simulink model "35 Bus Network Electricity Transmission Model"  (R2023b)
settings: Solver=VariableStepAuto  StartTime=0.0  StopTime=1  RelTol=1e-3
model workspace (MAT data in the model file):
  T_set = 0.0001
  Tp = 5e-05
undefined symbols (not defined in the file): D1, D11, Delta, DiscIntNeverNeededParam
libraries: spsSeriesRLCBranchLib x57, spsLoadFlowBusLib x35, spsThreePhaseSeriesRLCLoadLib x28, spsThreePhaseTransformerTwoWindingsLib x22, spsDistributedParametersLineLib x22, spsGenericPowerSystemStabilizerLib x20, spsThreePhaseVIMeasurementLib x14, spsSynchronousMachinepuStandardLib x10, spsExcitationSystemLib x10, spsHydraulicTurbineandGovernorLib x10, spsFourierLib x8, spsMeanLib x8
(part 5 of 8)

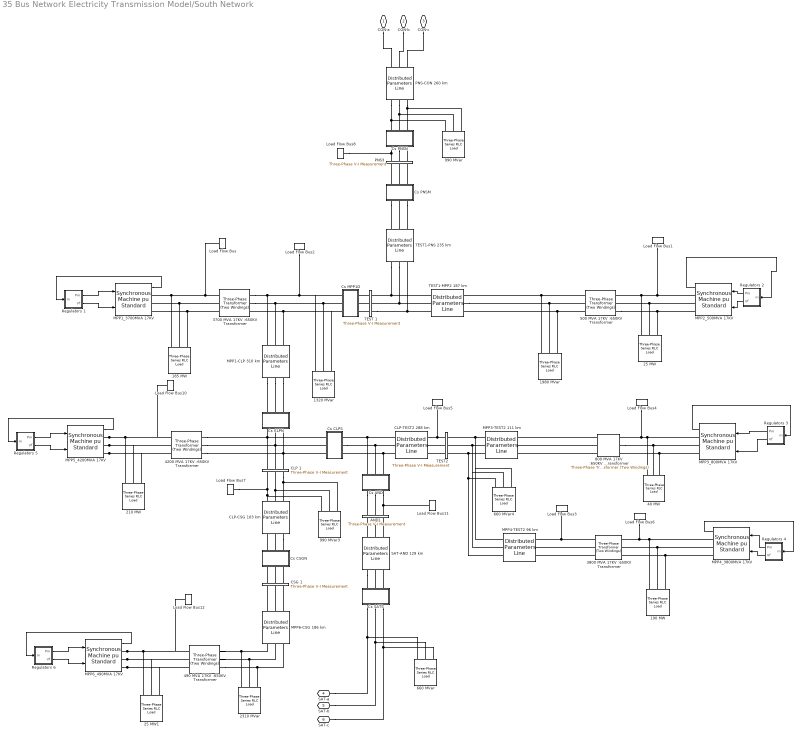
== system 35 Bus Network Electricity Transmission Model/South Network ==
  " SAT-AND 129 km" : spsDistributedParametersLineLib/Distributed Parameters Line  Phases=3  Length=129  Frequency=60  Resistance=[0.01273 0.3864]/6  Inductance="[0.9337e-3  4.1264e-3]/6"  Capacitance=[12.74e-9 7.751e-9]*6  x1=[-0.00078 2.90768445580107e-08 -136458.201500548 -192658.826474025;-0.00072 2.99535903710452e-08 -132065.820469422 -195695.922168478;-0.00066 3.08150113737671e-08 -127605.872124249 -198632.896213104;-0.0006 3.16606668472743e-08 -123080.638257011 -201468.245997714;-0.00054 3.24901241386005e-08 -118492.434060973 -204200.520904966;-0.00048 3.3302958882069e-08 -113843.60694618 -206828.323052531;-0.00042 3.40987552164055e-08 -109136.535338486 -209350.308008275;-0.00036 3.48771059975007e-08 -104373.627462701 -211765.185478092;-0.0003 3.56376130067127e-08 -99557.3201105034 -214071.719966049;-0.00024 3.63798871546032e-08 -94690.0773937295 -216268.73140648;-0.00018 3.71035486800023e-08 -89774.3894836895 -218355.095767737;-0.00012 3.7808227344302e-08 -84812.7713371497 -220329.745627261;-6e-05 3.84935626208767e-08 -79807.761409634 -222191.670717696]  x2=[-0.00078 6.20574629908019e-08 -60655.3196005387 -176454.698626756;-0.00072 6.44563826133641e-08 -56648.8312166304 -177781.461927132;-0.00066 6.68223251595644e-08 -52613.3602439216 -179017.268946562;-0.0006 6.91540801694784e-08 -48550.9713039289 -180161.487423341;-0.00054 7.14504546741573e-08 -44463.7427898983 -181213.531954152;-0.00048 7.37102738059722e-08 -40353.7658034608 -182172.864293574;-0.00042 7.59323813996988e-08 -36223.1430847865 -183038.993629456;-0.00036 7.81156405840321e-08 -32073.9879367833 -183811.476834026;-0.0003 8.02589343632316e-08 -27908.4231438924 -184489.918690602;-0.00024 8.23611661885963e-08 -23728.5798860328 -185073.972095794;-0.00018 8.44212605194795e-08 -19536.5966482498 -185563.338237088;-0.00012 8.64381633735555e-08 -15334.6181266266 -185957.766745723;-6e-05 8.84108428660558e-08 -11124.7941310188 -186257.055824787]  x3=[-0.00078 -1.45980787087981e-09 -866.244947874634 -13940.0125713573;-0.00072 -1.42091668020749e-09 -550.734822343354 -13956.0401157641;-0.00066 -1.38129852230606e-09 -234.942930700552 -13964.9274921696;-0.0006 -1.34097366655716e-09 80.9691620868421 -13966.670153628;-0.00054 -1.2999627439021e-09 396.839829554774 -13961.2672085614;-0.00048 -1.25828673628672e-09 712.50746643315 -13948.7214212164;-0.00042 -1.21596696592658e-09 1027.81057132607 -13929.0392102495;-0.00036 -1.17302508439819e-09 1342.58782933895 -13902.2306454436;-0.0003 -1.1294830615616e-09 1656.67819461017 -13868.3094425558;-0.00024 -1.08536317432028e-09 1969.92097270513 -13827.2929563003;-0.00018 -1.04068799522377e-09 2282.1559028305 -13779.2021714693;-0.00012 -9.95480380919198e-10 2593.22323982659 -13724.0616921971;-6e-05 -9.49763460457386e-10 2902.96383589593 -13661.8997293716]  x4=[-0.00078 2.00884929255157e-09 -4168.15373979615 6162.62143218946;-0.00072 1.99781306681485e-09 -4306.47032100265 6066.77150994181;-0.00066 1.9857547229978e-09 -4442.5836324185 5967.81771528863;-0.0006 1.97268043037194e-09 -4576.42403595849 5865.81067481971;-0.00054 1.95859687798696e-09 -4707.9230563991 5760.80257722184;-0.00048 1.94351127124849e-09 -4837.01341641164 5652.84714657807;-0.00042 1.92743132823169e-09 -4963.62907098261 5541.9996148815;-0.00036 1.91036527573254e-09 -5087.70524120354 5428.31669377758;-0.0003 1.89232184505882e-09 -5209.17844741309 5311.85654554936;-0.00024 1.87331026756309e-09 -5327.9865416744 5192.67875336062;-0.00018 1.85334026991968e-09 -5444.06873957111 5070.84429077198;-0.00012 1.83242206914838e-09 -5557.36565130583 4946.41549054576;-6e-05 1.81056636738724e-09 -5667.81931208504 4819.45601275533]  x5=0.000729548621424508  V1=[2.188e-18 3.182e-07 3.182e-07;377 377 377;0.6306 1.295 -0.2758]  V2=[1.209e-19 1.011e-07 1.011e-07;377 377 377;-2.255 -1.798 2.915]  I1=[1.016e-20 9.164e-09 9.164e-09;377 377 377;2.19 2.786 1.215]  I2=[1.089e-20 9.22e-09 9.22e-09;377 377 377;-0.7019 -0.2685 -1.839]  nHarmo=1  Measurements=None  Decoupling=off  VsMag0=0  VrMag0=0  VsAngle0=0  VrAngle0=0  IsMag0=0  IrMag0=0  IsAngle0=0  IrAngle0=0
      settings: LibrarySourceBlock=sps_lib/Power Grid Elements/Distributed Parameters Line
  1320 MVar : spsThreePhaseSeriesRLCLoadLib/Three-Phase Series RLC Load  LConnTagsString=A|B|C  Configuration=Y (grounded)  NominalVoltage=650e3  Vabc=[1e3 1e3 1e3]  Vabcp=[1e3 1e3 1e3]  NominalFrequency=60  UnbalancedPower=off  ActivePower=4400e3  InductivePower=1320e6  CapacitivePower=0  Pabc=[10e3 9e3 11e3]  QLabc=[100 90 110]  QCabc=[100 90 110]  Pabcp=[10e3 9e3 11e3]  QLabcp=[100 90 110]  QCabcp=[100 90 110]  Measurements=None  LoadType=constant Z
  185 MW : spsThreePhaseSeriesRLCLoadLib/Three-Phase Series RLC Load  LConnTagsString=A|B|C  Configuration=Y (grounded)  NominalVoltage=17e3  Vabc=[1e3 1e3 1e3]  Vabcp=[1e3 1e3 1e3]  NominalFrequency=60  UnbalancedPower=off  ActivePower=185e6  InductivePower=0  CapacitivePower=0  Pabc=[10e3 9e3 11e3]  QLabc=[100 90 110]  QCabc=[100 90 110]  Pabcp=[10e3 9e3 11e3]  QLabcp=[100 90 110]  QCabcp=[100 90 110]  Measurements=None  LoadType=constant Z
  190 MW : spsThreePhaseSeriesRLCLoadLib/Three-Phase Series RLC Load  LConnTagsString=A|B|C  Configuration=Y (grounded)  NominalVoltage=17e3  Vabc=[1e3 1e3 1e3]  Vabcp=[1e3 1e3 1e3]  NominalFrequency=60  UnbalancedPower=off  ActivePower=190e6  InductivePower=0  CapacitivePower=0  Pabc=[10e3 9e3 11e3]  QLabc=[100 90 110]  QCabc=[100 90 110]  Pabcp=[10e3 9e3 11e3]  QLabcp=[100 90 110]  QCabcp=[100 90 110]  Measurements=None  LoadType=constant Z
  1980 MVar : spsThreePhaseSeriesRLCLoadLib/Three-Phase Series RLC Load  LConnTagsString=A|B|C  Configuration=Y (grounded)  NominalVoltage=650e3  Vabc=[1e3 1e3 1e3]  Vabcp=[1e3 1e3 1e3]  NominalFrequency=60  UnbalancedPower=off  ActivePower=4400e3  InductivePower=1320e6  CapacitivePower=0  Pabc=[10e3 9e3 11e3]  QLabc=[100 90 110]  QCabc=[100 90 110]  Pabcp=[10e3 9e3 11e3]  QLabcp=[100 90 110]  QCabcp=[100 90 110]  Measurements=None  LoadType=constant Z
  210 MW : spsThreePhaseSeriesRLCLoadLib/Three-Phase Series RLC Load  LConnTagsString=A|B|C  Configuration=Y (grounded)  NominalVoltage=17e3  Vabc=[1e3 1e3 1e3]  Vabcp=[1e3 1e3 1e3]  NominalFrequency=60  UnbalancedPower=off  ActivePower=210e6  InductivePower=0  CapacitivePower=0  Pabc=[10e3 9e3 11e3]  QLabc=[100 90 110]  QCabc=[100 90 110]  Pabcp=[10e3 9e3 11e3]  QLabcp=[100 90 110]  QCabcp=[100 90 110]  Measurements=None  LoadType=constant Z
  2310 MVar : spsThreePhaseSeriesRLCLoadLib/Three-Phase Series RLC Load  LConnTagsString=A|B|C  Configuration=Y (grounded)  NominalVoltage=650e3  Vabc=[1e3 1e3 1e3]  Vabcp=[1e3 1e3 1e3]  NominalFrequency=60  UnbalancedPower=off  ActivePower=7700e3  InductivePower=2310e6  CapacitivePower=0  Pabc=[10e3 9e3 11e3]  QLabc=[100 90 110]  QCabc=[100 90 110]  Pabcp=[10e3 9e3 11e3]  QLabcp=[100 90 110]  QCabcp=[100 90 110]  Measurements=None  LoadType=constant Z
  25 MW : spsThreePhaseSeriesRLCLoadLib/Three-Phase Series RLC Load  LConnTagsString=A|B|C  Configuration=Y (grounded)  NominalVoltage=17e3  Vabc=[1e3 1e3 1e3]  Vabcp=[1e3 1e3 1e3]  NominalFrequency=60  UnbalancedPower=off  ActivePower=25e6  InductivePower=0  CapacitivePower=0  Pabc=[10e3 9e3 11e3]  QLabc=[100 90 110]  QCabc=[100 90 110]  Pabcp=[10e3 9e3 11e3]  QLabcp=[100 90 110]  QCabcp=[100 90 110]  Measurements=None  LoadType=constant Z
  25 MW1 : spsThreePhaseSeriesRLCLoadLib/Three-Phase Series RLC Load  LConnTagsString=A|B|C  Configuration=Y (grounded)  NominalVoltage=17e3  Vabc=[1e3 1e3 1e3]  Vabcp=[1e3 1e3 1e3]  NominalFrequency=60  UnbalancedPower=off  ActivePower=25e6  InductivePower=0  CapacitivePower=0  Pabc=[10e3 9e3 11e3]  QLabc=[100 90 110]  QCabc=[100 90 110]  Pabcp=[10e3 9e3 11e3]  QLabcp=[100 90 110]  QCabcp=[100 90 110]  Measurements=None  LoadType=constant Z
  "3700 MVA 17KV :650KV Transformer " : spsThreePhaseTransformerTwoWindingsLib/Three-Phase Transformer (Two Windings)  Winding1Connection=Delta (D1)  Winding2Connection=Yg  CoreType=Three single-phase transformers  SetSaturation=off  Hysteresis=off  DataFile='hysteresis'  SetInitialFlux=off  Measurements=None  UNITS=pu  NominalPower=[ 3700e6 , 60 ]  Winding1=[ 17e3 , 0.002 , 0.08 ]  Winding2=[ 650e3 , 0.002 , 0.08 ]  Rm=500  Lm=500  L0=0.5  Saturation=[ 0,0 ; 0.0024,1.2 ; 1.0,1.52 ]  InitialFluxes=[ 0.8 , -0.8 , 0.7 ]  BreakLoop=off  DiscreteSolver=Trapezoidal iterative  DataType=off  TransfoNumber=1
  3800 MVA 17KV :650KV Transformer : spsThreePhaseTransformerTwoWindingsLib/Three-Phase Transformer (Two Windings)  Winding1Connection=Yg  Winding2Connection=Delta (D1)  CoreType=Three single-phase transformers  SetSaturation=off  Hysteresis=off  DataFile='hysteresis'  SetInitialFlux=off  Measurements=None  UNITS=pu  NominalPower=[ 3800e6 , 60 ]  Winding1=[ 650e3 , 0.002 , 0.08 ]  Winding2=[ 17e3 , 0.002 , 0.08 ]  Rm=500  Lm=500  L0=0.5  Saturation=[ 0,0 ; 0.0024,1.2 ; 1.0,1.52 ]  InitialFluxes=[ 0.8 , -0.8 , 0.7 ]  BreakLoop=off  DiscreteSolver=Trapezoidal iterative  DataType=off  TransfoNumber=1
  40 MW : spsThreePhaseSeriesRLCLoadLib/Three-Phase Series RLC Load  LConnTagsString=A|B|C  Configuration=Y (grounded)  NominalVoltage=17e3  Vabc=[1e3 1e3 1e3]  Vabcp=[1e3 1e3 1e3]  NominalFrequency=60  UnbalancedPower=off  ActivePower=40e6  InductivePower=0  CapacitivePower=0  Pabc=[10e3 9e3 11e3]  QLabc=[100 90 110]  QCabc=[100 90 110]  Pabcp=[10e3 9e3 11e3]  QLabcp=[100 90 110]  QCabcp=[100 90 110]  Measurements=None  LoadType=constant Z
  4200 MVA 17KV :650KV Transformer : spsThreePhaseTransformerTwoWindingsLib/Three-Phase Transformer (Two Windings)  Winding1Connection=Delta (D1)  Winding2Connection=Yg  CoreType=Three single-phase transformers  SetSaturation=off  Hysteresis=off  DataFile='hysteresis'  SetInitialFlux=off  Measurements=None  UNITS=pu  NominalPower=[ 4200e6 , 60 ]  Winding1=[ 17e3 , 0.002 , 0.08 ]  Winding2=[ 650e3 , 0.002 , 0.08 ]  Rm=500  Lm=500  L0=0.5  Saturation=[ 0,0 ; 0.0024,1.2 ; 1.0,1.52 ]  InitialFluxes=[ 0.8 , -0.8 , 0.7 ]  BreakLoop=off  DiscreteSolver=Trapezoidal iterative  DataType=off  TransfoNumber=1
  490 MVA 17KV :650KV Transformer : spsThreePhaseTransformerTwoWindingsLib/Three-Phase Transformer (Two Windings)  Winding1Connection=Delta (D1)  Winding2Connection=Yg  CoreType=Three single-phase transformers  SetSaturation=off  Hysteresis=off  DataFile='hysteresis'  SetInitialFlux=off  Measurements=None  UNITS=pu  NominalPower=[ 490e6 , 60 ]  Winding1=[ 17e3 , 0.002 , 0.08 ]  Winding2=[ 650e3 , 0.002 , 0.08 ]  Rm=500  Lm=500  L0=0.5  Saturation=[ 0,0 ; 0.0024,1.2 ; 1.0,1.52 ]  InitialFluxes=[ 0.8 , -0.8 , 0.7 ]  BreakLoop=off  DiscreteSolver=Trapezoidal iterative  DataType=off  TransfoNumber=1
  "500 MVA 17KV :650KV Transformer " : spsThreePhaseTransformerTwoWindingsLib/Three-Phase Transformer (Two Windings)  Winding1Connection=Yg  Winding2Connection=Delta (D1)  CoreType=Three single-phase transformers  SetSaturation=off  Hysteresis=off  DataFile='hysteresis'  SetInitialFlux=off  Measurements=None  UNITS=pu  NominalPower=[ 500e6 , 60 ]  Winding1=[650e3 , 0.002 , 0.08 ]  Winding2=[17e3 , 0.002 , 0.08 ]  Rm=500  Lm=500  L0=0.5  Saturation=[ 0,0 ; 0.0024,1.2 ; 1.0,1.52 ]  InitialFluxes=[ 0.8 , -0.8 , 0.7 ]  BreakLoop=off  DiscreteSolver=Trapezoidal iterative  DataType=off  TransfoNumber=1
  660 MVar : spsThreePhaseSeriesRLCLoadLib/Three-Phase Series RLC Load  LConnTagsString=A|B|C  Configuration=Y (grounded)  NominalVoltage=650e3  Vabc=[1e3 1e3 1e3]  Vabcp=[1e3 1e3 1e3]  NominalFrequency=60  UnbalancedPower=off  ActivePower=2200e3  InductivePower=660e6  CapacitivePower=0  Pabc=[10e3 9e3 11e3]  QLabc=[100 90 110]  QCabc=[100 90 110]  Pabcp=[10e3 9e3 11e3]  QLabcp=[100 90 110]  QCabcp=[100 90 110]  Measurements=None  LoadType=constant Z
  660 MVar4 : spsThreePhaseSeriesRLCLoadLib/Three-Phase Series RLC Load  LConnTagsString=A|B|C  Configuration=Y (grounded)  NominalVoltage=650e3  Vabc=[1e3 1e3 1e3]  Vabcp=[1e3 1e3 1e3]  NominalFrequency=60  UnbalancedPower=off  ActivePower=2200e3  InductivePower=660e6  CapacitivePower=0  Pabc=[10e3 9e3 11e3]  QLabc=[100 90 110]  QCabc=[100 90 110]  Pabcp=[10e3 9e3 11e3]  QLabcp=[100 90 110]  QCabcp=[100 90 110]  Measurements=None  LoadType=constant Z
  800 MVA 17KV :650KV Transformer : spsThreePhaseTransformerTwoWindingsLib/Three-Phase Transformer (Two Windings)  Winding1Connection=Yg  Winding2Connection=Delta (D1)  CoreType=Three single-phase transformers  SetSaturation=off  Hysteresis=off  DataFile='hysteresis'  SetInitialFlux=off  Measurements=None  UNITS=pu  NominalPower=[ 800e6 , 60 ]  Winding1=[650e3 , 0.002 , 0.08 ]  Winding2=[ 17e3 , 0.002 , 0.08 ]  Rm=500  Lm=500  L0=0.5  Saturation=[ 0,0 ; 0.0024,1.2 ; 1.0,1.52 ]  InitialFluxes=[ 0.8 , -0.8 , 0.7 ]  BreakLoop=off  DiscreteSolver=Trapezoidal iterative  DataType=off  TransfoNumber=1
  990 MVar : spsThreePhaseSeriesRLCLoadLib/Three-Phase Series RLC Load  LConnTagsString=A|B|C  Configuration=Y (grounded)  NominalVoltage=650e3  Vabc=[1e3 1e3 1e3]  Vabcp=[1e3 1e3 1e3]  NominalFrequency=60  UnbalancedPower=off  ActivePower=2200e3  InductivePower=660e6  CapacitivePower=0  Pabc=[10e3 9e3 11e3]  QLabc=[100 90 110]  QCabc=[100 90 110]  Pabcp=[10e3 9e3 11e3]  QLabcp=[100 90 110]  QCabcp=[100 90 110]  Measurements=None  LoadType=constant Z
  990 MVar3 : spsThreePhaseSeriesRLCLoadLib/Three-Phase Series RLC Load  LConnTagsString=A|B|C  Configuration=Y (grounded)  NominalVoltage=650e3  Vabc=[1e3 1e3 1e3]  Vabcp=[1e3 1e3 1e3]  NominalFrequency=60  UnbalancedPower=off  ActivePower=3300e3  InductivePower=990e6  CapacitivePower=0  Pabc=[10e3 9e3 11e3]  QLabc=[100 90 110]  QCabc=[100 90 110]  Pabcp=[10e3 9e3 11e3]  QLabcp=[100 90 110]  QCabcp=[100 90 110]  Measurements=None  LoadType=constant Z
  AND1 : spsThreePhaseVIMeasurementLib/Three-Phase V-I Measurement  VoltageMeasurement=no  SetLabelV=off  LabelV=Vabc  Vpu=off  VpuLL=off  CurrentMeasurement=no  SetLabelI=off  LabelI=Iabc  Ipu=off  Pbase=100e6  Vbase=500e3  OutputType=Complex  PhasorSimulation=off  PSBequivalent=0
  CLP 1 : spsThreePhaseVIMeasurementLib/Three-Phase V-I Measurement  VoltageMeasurement=no  SetLabelV=off  LabelV=Vabc  Vpu=off  VpuLL=off  CurrentMeasurement=no  SetLabelI=off  LabelI=Iabc  Ipu=off  Pbase=100e6  Vbase=500e3  OutputType=Complex  PhasorSimulation=off  PSBequivalent=0
  CLP-CSG 103 km : spsDistributedParametersLineLib/Distributed Parameters Line  Phases=3  Length=103  Frequency=60  Resistance=[0.01273 0.3864]/6  Inductance="[0.9337e-3  4.1264e-3]/6"  Capacitance=[12.74e-9 7.751e-9]*6  x1=[-0.0006 5.12425584959224e-09 -127463.751672335 -207117.664561966;-0.00054 6.49412639945238e-09 -122746.650233849 -209947.630266697;-0.00048 7.8606744342489e-09 -117966.749341006 -212670.182884398;-0.00042 9.2232008027563e-09 -113126.494479425 -215283.929506842;-0.00036 1.05810084113079e-08 -108228.362012931 -217787.53289296;-0.0003 1.19334025804416e-08 -103274.857916601 -220179.712153;-0.00024 1.32796914003113e-08 -98268.5164946604 -222459.243403849;-0.00018 1.46191860846801e-08 -93211.8990838882 -224624.960395198;-0.00012 1.59512013233165e-08 -88107.5927431868 -226675.755106218;-6e-05 1.72750556326116e-08 -82958.2089299969 -228610.578312438]  x2=[-0.0006 1.03580737650098e-09 -130162.098088271 -208255.374210334;-0.00054 2.56309005743374e-09 -125418.574057825 -211146.078979345;-0.00048 4.08906141413265e-09 -120610.883567423 -213928.75751282;-0.00042 5.61294073145493e-09 -115741.486320354 -216601.986141002;-0.00036 7.13394836458377e-09 -110812.873590228 -219164.39719073;-0.0003 8.65130613790908e-09 -105827.566946386 -221614.679685162;-0.00024 1.01642377431565e-08 -100788.116963826 -223951.5800145;-0.00018 1.1671969136561e-08 -95697.1019182766 -226173.902577352;-0.00012 1.3173728934882e-08 -90557.1264671069 -228280.510392433;-6e-05 1.46687488100574e-08 -85370.8203167333 -230270.325680258]  x3=[-0.0006 -2.87618472727126e-10 -3326.0649498337 -3945.27936955612;-0.00054 -2.78422639605714e-10 -3235.98145838752 -4019.4982124491;-0.00048 -2.69084360317222e-10 -3144.24237903318 -4091.6606057848;-0.00042 -2.59608412497884e-10 -3050.8946471788 -4161.72962994939;-0.00036 -2.499996442177e-10 -2955.98602124887 -4229.66943633538;-0.0003 -2.40262971500072e-10 -2859.56505825013 -4295.44526568243;-0.00024 -2.30403375806675e-10 -2761.6810889289 -4359.02346586085;-0.00018 -2.20425901488851e-10 -2662.38419253258 -4420.37150908865;-0.00012 -2.10335653206822e-10 -2561.72517118816 -4479.45800857332;-6e-05 -2.00137793318057e-10 -2459.75552391091 -4536.25273456994]  x4=[-0.0006 2.22700166548668e-10 -2978.89511835108 -4845.29955542766;-0.00054 2.36457740037183e-10 -2868.544242262 -4911.43608496111;-0.00048 2.50094337376658e-10 -2756.72576593397 -4975.05983304058;-0.00042 2.63602981831919e-10 -2643.49689776566 -5036.13824858094;-0.00036 2.76976762130852e-10 -2528.91556773825 -5094.64008273619;-0.0003 2.90208836000337e-10 -2413.04039777739 -5150.53540488699;-0.00024 3.03292433666881e-10 -2295.93067176117 -5203.79561795369;-0.00018 3.16220861320161e-10 -2177.64630518935 -5254.39347302716;-0.00012 3.28987504537701e-10 -2058.24781452953 -5302.3030833098;-6e-05 3.41585831668928e-10 -1937.79628625574 -5347.49993735973]  x5=0.000582507814005615  V1=[1.056e-22 6.221e-12 6.221e-12;377 377 377;0.3647 1.373 -0.1974]  V2=[1.588e-22 9.824e-12 9.824e-12;377 377 377;0.3755 1.375 -0.1957]  I1=[3.913e-25 1.044e-13 1.044e-13;377 377 377;-0.5956 0.0636 -1.507]  I2=[3.097e-25 1.021e-13 1.021e-13;377 377 377;1.525 2.624 1.053]  nHarmo=1  Measurements=None  Decoupling=off  VsMag0=0  VrMag0=0  VsAngle0=0  VrAngle0=0  IsMag0=0  IrMag0=0  IsAngle0=0  IrAngle0=0
      settings: LibrarySourceBlock=sps_lib/Power Grid Elements/Distributed Parameters Line
  CLP-TEST2 288 km : spsDistributedParametersLineLib/Distributed Parameters Line  Phases=3  Length=288  Frequency=60  Resistance=[0.01273 0.3864]/6  Inductance="[0.9337e-3  4.1264e-3]/6"  Capacitance=[12.74e-9 7.751e-9]*6  x1=[-0.00168 -9.01889044932841e-09 0 0;-0.00162 -8.63227494376247e-09 0 0;-0.00156 -8.2412430068292e-09 0 0;-0.0015 -7.84599469769297e-09 0 0;-0.00144 -7.4467322326921e-09 0 0;-0.00138 -7.04365988188118e-09 0 0;-0.00132 -6.63698386452283e-09 0 0;-0.00126 -6.22691224358202e-09 0 0;-0.0012 -5.81365481927729e-09 0 0;-0.00114 -5.39742302174303e-09 0 0;-0.00108 -4.97842980285793e-09 0 0;-0.00102 -4.55688952729489e-09 -44206.8856372299 -153787.637229117;-0.00096 -4.13301786284804e-09 -40717.2774853985 -154748.172851438;-0.0009 -3.70703167009317e-09 -37206.8376220368 -155629.53644911;-0.00084 -3.27914889143781e-09 -33677.3620530444 -156431.277100231;-0.00078 -2.84958843961789e-09 -30130.6565233395 -157152.98461947;-0.00072 -2.41857008569792e-09 -26568.5355930067 -157794.289767925;-0.00066 -1.98631434663207e-09 -22992.8217089345 -158354.864442031;-0.0006 -1.55304237244361e-09 -19405.3442724175 -158834.421841427;-0.00054 -1.11897583308049e-09 -15807.9387032012 -159232.716615686;-0.00048 -6.84336805004866e-10 -12202.4455004472 -159549.544989843;-0.00042 -2.49347657574712e-10 -8590.70930109991 -159784.744868646;-0.00036 1.85769060724472e-10 -4974.57793613612 -159938.195919491;-0.0003 6.20790736139571e-10 -1355.90148518057 -160009.819633986;-0.00024 1.05549480354317e-09 2263.46867002897 -159999.579368115;-0.00018 1.48965886030197e-09 5881.68079284284 -159907.480360987;-0.00012 1.92306078006211e-09 9496.88373908212 -159733.569732156;-6e-05 2.3554788263931e-09 13107.2279041183 -159477.936457512]  x2=[-0.00168 4.60556142135583e-08 0 0;-0.00162 4.54395735280648e-08 0 0;-0.00156 4.48002851171275e-08 0 0;-0.0015 4.41380760525103e-08 0 0;-0.00144 4.34532851326066e-08 0 0;-0.00138 4.27462627091048e-08 0 0;-0.00132 4.20173705077409e-08 0 0;-0.00126 4.12669814432335e-08 0 0;-0.0012 4.04954794284935e-08 0 0;-0.00114 3.97032591782076e-08 0 0;-0.00108 3.88907260068941e-08 0 0;-0.00102 3.80582956215376e-08 -131291.493502831 -180468.685421767;-0.00096 3.72063939089046e-08 -127176.143665401 -183392.040265848;-0.0009 3.63354567176528e-08 -122995.728162927 -186221.568353434;-0.00084 3.54459296353421e-08 -118752.385773224 -188955.822045672;-0.00078 3.45382677604645e-08 -114448.287468669 -191593.402447849;-0.00072 3.36129354696069e-08 -110085.635305483 -194132.960125094;-0.00066 3.26704061798673e-08 -105666.661297126 -196573.195792775;-0.0006 3.17111621066465e-08 -101193.626272354 -198912.860981233;-0.00054 3.0735694016937e-08 -96668.818718538 -201150.758674526;-0.00048 2.97445009782381e-08 -92094.5536108312 -203285.743922843;-0.00042 2.87380901032235e-08 -87473.1712277854 -205316.72442828;-0.00036 2.77169762902933e-08 -82807.0359540211 -207242.661103682;-0.0003 2.66816819601421e-08 -78098.5350705646 -209062.56860426;-0.00024 2.56327367884793e-08 -73350.077533471 -210775.515831708;-0.00018 2.45706774350371e-08 -68564.0927413577 -212380.626410572;-0.00012 2.34960472690051e-08 -63743.0292924792 -213877.079136623;-6e-05 2.24093960910333e-08 -58889.3537319788 -215264.108396992]  x3=[-0.00168 5.97743378198794e-10 0 0;-0.00162 6.126895975751e-10 0 0;-0.00156 6.27322353632085e-10 0 0;-0.0015 6.41634159981367e-10 0 0;-0.00144 6.55617694438366e-10 0 0;-0.00138 6.69265802768469e-10 0 0;-0.00132 6.82571502347266e-10 0 0;-0.00126 6.9552798573299e-10 0 0;-0.0012 7.08128624149334e-10 0 0;-0.00114 7.2036697087685e-10 0 0;-0.00108 7.32236764551215e-10 0 0;-0.00102 7.43731932366655e-10 -3398.58946063306 1988.93086529394;-0.00096 7.54846593182911e-10 -3442.70433280188 1911.55410097375;-0.0009 7.65575060534133e-10 -3485.05785382017 1833.19935025405;-0.00084 7.75911845538185e-10 -3525.62835484399 1753.90670087312;-0.00078 7.85851659704858e-10 -3564.39507925535 1673.71672041556;-0.00072 7.95389417641556e-10 -3601.33819328171 1592.67043555711;-0.00066 8.04520239655082e-10 -3636.43879614331 1510.80931107466;-0.0006 8.13239454248176e-10 -3669.67892972315 1428.17522863212;-0.00054 8.21542600509539e-10 -3701.04158775466 1344.81046535296;-0.00048 8.2942543039612e-10 -3730.51072452249 1260.75767219049;-0.00042 8.3688391090649e-10 -3758.07126307175 1176.05985210681;-0.00036 8.43914226144203e-10 -3783.70910292164 1090.7603380717;-0.0003 8.5051277927008e-10 -3807.41112727958 1004.9027708927;-0.00024 8.56676194342412e-10 -3829.16520975193 918.531076887637;-0.00018 8.62401318044163e-10 -3848.96022054813 831.689445411139;-0.00012 8.67685221296259e-10 -3866.78603217489 744.422306246515;-6e-05 8.72525200756159e-10 -3882.6335246176 656.774306874673]  x4=[-0.00168 -3.02423306475975e-10 0 0;-0.00162 -3.17054030089913e-10 0 0;-0.00156 -3.31522543003572e-10 0 0;-0.0015 -3.45821442858398e-10 0 0;-0.00144 -3.59943414073012e-10 0 0;-0.00138 -3.73881231585997e-10 0 0;-0.00132 -3.87627764552372e-10 0 0;-0.00126 -4.01175979991864e-10 0 0;-0.0012 -4.14518946387112e-10 0 0;-0.00114 -4.2764983722996e-10 0 0;-0.00108 -4.4056193451402e-10 0 0;-0.00102 -4.53248632171734e-10 -1845.28470206776 -8589.47178879478;-0.00096 -4.65703439454157e-10 -1650.53999099367 -8629.01124032957;-0.0009 -4.77919984251745e-10 -1454.95083316171 -8664.13593026801;-0.00084 -4.89892016354445e-10 -1258.61729559911 -8694.82788816971;-0.00078 -5.01613410649413e-10 -1061.6398261715 -8721.07141146187;-0.00072 -5.13078170254743e-10 -864.119202191978 -8742.85307347305;-0.00066 -5.24280429587577e-10 -666.156478861526 -8760.1617303025;-0.0006 -5.35214457365045e-10 -467.852937567331 -8772.98852652155;-0.00054 -5.45874659536499e-10 -269.310034065349 -8781.32689970423;-0.00048 -5.5625558214553e-10 -70.6293465736623 -8785.17258378477;-0.00042 -5.66351914120313e-10 128.087476196812 -8784.52361124011;-0.00036 -5.76158489990853e-10 326.73876704768 -8779.38031409662;-0.0003 -5.85670292531729e-10 525.222892307888 -8769.74532376013;-0.00024 -5.94882455329003e-10 723.438303831388 -8755.62356966975;-0.00018 -6.03790265269966e-10 921.283590951045 -8737.0222767758;-0.00012 -6.12389164954456e-10 1118.65753236221 -8713.95096184344;-6e-05 -6.20674755026505e-10 1315.4591479094 -8686.4214285837]  x5=0.00162875971294774  V1=[1.245e-23 7.93e-13 7.93e-13;377 377 377;-1.837 -1.972 2.74]  V2=[6.065e-20 5.187e-08 5.187e-08;377 377 377;-2.594 -2.004 2.709]  I1=[1.297e-22 5.199e-10 5.199e-10;377 377 377;2.342 2.744 1.173]  I2=[1.117e-22 5.13e-10 5.13e-10;377 377 377;-1.44 -0.7735 -2.344]  nHarmo=1  Measurements=None  Decoupling=off  VsMag0=0  VrMag0=0  VsAngle0=0  VrAngle0=0  IsMag0=0  IrMag0=0  IsAngle0=0  IrAngle0=0
      settings: LibrarySourceBlock=sps_lib/Power Grid Elements/Distributed Parameters Line
  CSG 1 : spsThreePhaseVIMeasurementLib/Three-Phase V-I Measurement  VoltageMeasurement=no  SetLabelV=off  LabelV=Vabc  Vpu=off  VpuLL=off  CurrentMeasurement=no  SetLabelI=off  LabelI=Iabc  Ipu=off  Pbase=100e6  Vbase=500e3  OutputType=Complex  PhasorSimulation=off  PSBequivalent=0
  Cs AND : Subsystem
  Cs CLPN : Subsystem
  Cs CLPS : Subsystem
  Cs CSGN : Subsystem
  Cs MPP1D : Subsystem
  Cs PNSM : Subsystem
  Cs PNSN : Subsystem
  Cs SATS : Subsystem
  Load Flow Bus : spsLoadFlowBusLib/Load Flow Bus  LConnTagsString=a  Phases=single  Connectors=on one side  ID=BUS_1  Vbase=17e3  Vref=1  Vangle=0  VLF=1  VLFb=1  VLFc=1  angleLF=0  angleLFb=0  angleLFc=0
  Load Flow Bus1 : spsLoadFlowBusLib/Load Flow Bus  LConnTagsString=a  Phases=single  Connectors=on one side  ID=BUS_2  Vbase=17e3  Vref=1  Vangle=0  VLF=1  VLFb=1  VLFc=1  angleLF=0  angleLFb=0  angleLFc=0
  Load Flow Bus10 : spsLoadFlowBusLib/Load Flow Bus  LConnTagsString=a  Phases=single  Connectors=on one side  ID=BUS_5  Vbase=17e3  Vref=1  Vangle=0  VLF=1  VLFb=1  VLFc=1  angleLF=0  angleLFb=0  angleLFc=0
  Load Flow Bus11 : spsLoadFlowBusLib/Load Flow Bus  LConnTagsString=a  Phases=single  Connectors=on one side  ID=BUS_11  Vbase=650e3  Vref=1.031  Vangle=17.31  VLF=1  VLFb=1  VLFc=1  angleLF=0  angleLFb=0  angleLFc=0
  Load Flow Bus12 : spsLoadFlowBusLib/Load Flow Bus  LConnTagsString=a  Phases=single  Connectors=on one side  ID=BUS_6  Vbase=17e3  Vref=1  Vangle=0  VLF=1  VLFb=1  VLFc=1  angleLF=0  angleLFb=0  angleLFc=0
  Load Flow Bus2 : spsLoadFlowBusLib/Load Flow Bus  LConnTagsString=a  Phases=single  Connectors=on one side  ID=BUS_7  Vbase=650e3  Vref=1  Vangle=0  VLF=1  VLFb=1  VLFc=1  angleLF=0  angleLFb=0  angleLFc=0
  Load Flow Bus3 : spsLoadFlowBusLib/Load Flow Bus  LConnTagsString=a  Phases=single  Connectors=on one side  ID=BUS_9  Vbase=650e3  Vref=1.031  Vangle=17.31  VLF=1  VLFb=1  VLFc=1  angleLF=0  angleLFb=0  angleLFc=0
  Load Flow Bus4 : spsLoadFlowBusLib/Load Flow Bus  LConnTagsString=a  Phases=single  Connectors=on one side  ID=BUS_3  Vbase=17e3  Vref=1  Vangle=0  VLF=1  VLFb=1  VLFc=1  angleLF=0  angleLFb=0  angleLFc=0
  Load Flow Bus5 : spsLoadFlowBusLib/Load Flow Bus  LConnTagsString=a  Phases=single  Connectors=on one side  ID=BUS_8  Vbase=650e3  Vref=1.031  Vangle=17.31  VLF=1  VLFb=1  VLFc=1  angleLF=0  angleLFb=0  angleLFc=0
  Load Flow Bus6 : spsLoadFlowBusLib/Load Flow Bus  LConnTagsString=a  Phases=single  Connectors=on one side  ID=BUS_4  Vbase=17e3  Vref=1  Vangle=0  VLF=1  VLFb=1  VLFc=1  angleLF=0  angleLFb=0  angleLFc=0
  Load Flow Bus7 : spsLoadFlowBusLib/Load Flow Bus  LConnTagsString=a  Phases=single  Connectors=on one side  ID=BUS_10  Vbase=650e3  Vref=1.031  Vangle=17.31  VLF=1  VLFb=1  VLFc=1  angleLF=0  angleLFb=0  angleLFc=0
  Load Flow Bus8 : spsLoadFlowBusLib/Load Flow Bus  LConnTagsString=a  Phases=single  Connectors=on one side  ID=BUS_12  Vbase=650e3  Vref=1  Vangle=0  VLF=1  VLFb=1  VLFc=1  angleLF=0  angleLFb=0  angleLFc=0
  MPP1-CLP 310 km : spsDistributedParametersLineLib/Distributed Parameters Line  Phases=3  Length=310  Frequency=60  Resistance=[0.01273 0.3864]/6  Inductance="[0.9337e-3  4.1264e-3]/6"  Capacitance=[12.74e-9 7.751e-9]*6  x1=[-0.0018 1.412401861212e-08 -201242.370163828 -148550.970561651;-0.00174 1.28123826835698e-08 -197831.016179838 -153064.605828986;-0.00168 1.1494191703293e-08 -194318.448192473 -157499.930415671;-0.00162 1.01701200821527e-08 -190706.46329642 -161854.675127691;-0.00156 8.84084523965606e-09 -186996.909449895 -166126.611997184;-0.0015 7.5070472573748e-09 -183191.68452919 -170313.555422314;-0.00144 6.16940853100238e-09 -179292.735357687 -174413.363285456;-0.00138 4.82861342122793e-09 -175302.056709825 -178423.938049153;-0.00132 3.48534790360467e-09 -171221.690290542 -182343.22782925;-0.00126 2.1402992175921e-09 -167053.723690692 -186169.227444673;-0.0012 7.94155514951635e-10 -162800.289319005 -189899.979443323;-0.00114 -5.52394492324591e-10 -158463.563311099 -193533.575103543;-0.00108 -1.89866188437147e-09 -154045.764416132 -197068.15541065;-0.00102 -3.24395788591506e-09 -149549.152861652 -200501.912008048;-0.00096 -4.58759421866277e-09 -144976.029197217 -203833.088122413;-0.0009 -5.92888345343922e-09 -140328.733117396 -207059.979462493;-0.00084 -7.26713936188772e-09 -135609.642264735 -210180.935091051;-0.00078 -8.60167726755738e-09 -130821.171013314 -213194.358269519;-0.00072 -9.93181439619624e-09 -125965.769233504 -216098.707274918;-0.00066 -1.12568702250712e-08 -121045.921038576 -218892.49618863;-0.0006 -1.25761668311359e-08 -116064.143513772 -221574.295656623;-0.00054 -1.3889029237869e-08 -111022.985428528 -224142.733620737;-0.00048 -1.51947857606042e-08 -105925.025932469 -226596.496020648;-0.00042 -1.6492768350177e-08 -100772.873235875 -228934.327466174;-0.00036 -1.77823129347105e-08 -95569.1632752638 -231155.031879547;-0.0003 -1.90627597593672e-08 -90316.5583648063 -233257.473107358;-0.00024 -2.03334537238917e-08 -85017.7458342311 -235240.575501824;-0.00018 -2.15937447177721e-08 -79675.4366539399 -237103.324471117;-0.00012 -2.28429879528483e-08 -74292.3640480237 -238844.766998445;-6e-05 -2.4080544293198e-08 -68871.2820958955 -240464.012129633]  x2=[-0.0018 8.50892791491867e-08 -204438.071485386 -118555.914824297;-0.00174 8.56840691370501e-08 -201704.31469779 -123149.498911936;-0.00168 8.62350215718834e-08 -198867.362255727 -127680.077440391;-0.00162 8.67418545762406e-08 -195928.665596487 -132145.332481971;-0.00156 8.72043088449914e-08 -192889.728211583 -136542.979529688;-0.0015 8.76221477779866e-08 -189752.104877533 -140870.768666053;-0.00144 8.79951576011076e-08 -186517.400860412 -145126.485714177;-0.00138 8.83231474756362e-08 -183187.271094566 -149307.95337058;-0.00132 8.86059495958923e-08 -179763.419335916 -153413.032319145;-0.00126 8.88434192750853e-08 -176247.597290288 -157439.622325628;-0.0012 8.90354350193396e-08 -172641.603717205 -161385.66331218;-0.00114 8.91818985898523e-08 -168947.28350961 -165249.136411317;-0.00108 8.92827350531544e-08 -165166.526749985 -169028.064998813;-0.00102 8.9337892819448e-08 -161301.267743348 -172720.515704976;-0.00096 8.93473436690008e-08 -157353.484027629 -176324.599403797;-0.0009 8.93110827665834e-08 -153325.195361923 -179838.472179458;-0.00084 8.92291286639436e-08 -149218.462693146 -183260.33626972;-0.00078 8.91015232903146e-08 -145035.387101616 -186588.440985684;-0.00072 8.89283319309634e-08 -140778.108726098 -189821.083607482;-0.00066 8.87096431937896e-08 -136448.805668875 -192956.610255416;-0.0006 8.84455689639922e-08 -132049.692881389 -195993.416736115;-0.00054 8.81362443468266e-08 -127583.021031026 -198929.94936327;-0.00048 8.77818275984827e-08 -123051.075349641 -201764.705752528;-0.00042 8.73825000451176e-08 -118456.174464384 -204496.23559014;-0.00036 8.69384659900866e-08 -113800.669211453 -207123.141374968;-0.0003 8.64499526094168e-08 -109086.941433359 -209644.079133473;-0.00024 8.59172098355806e-08 -104317.402760333 -212057.759107316;-0.00018 8.5340510229625e-08 -99494.49337649 -214362.946413223;-0.00012 8.47201488417247e-08 -94620.6807713891 -216558.461674773;-6e-05 8.40564430602285e-08 -89698.4584776165 -218643.18162579]  x3=[-0.0018 -5.53738536744532e-10 -3404.66204910686 -2113.73097377968;-0.00174 -5.38456820191621e-10 -3355.98338351194 -2190.19590865274;-0.00168 -5.22899619179961e-10 -3305.58773480657 -2265.54029882876;-0.00162 -5.07074893061054e-10 -3253.50088633584 -2339.72559672553;-0.00156 -4.90990738057191e-10 -3199.74948669387 -2412.71384777386;-0.0015 -4.74655383119272e-10 -3144.36103608993 -2484.46770983584;-0.00144 -4.58077185716726e-10 -3087.36387227882 -2554.95047230979;-0.00138 -4.41264627561675e-10 -3028.78715606273 -2624.12607491204;-0.00132 -4.24226310269529e-10 -2968.66085637204 -2691.9591261261;-0.00126 -4.06970950958249e-10 -2907.01573493269 -2758.41492130954;-0.0012 -3.89507377788501e-10 -2843.88333052787 -2823.45946044959;-0.00114 -3.71844525447007e-10 -2779.29594286223 -2887.05946555815;-0.00108 -3.53991430575397e-10 -2713.28661603674 -2949.1823976974;-0.00102 -3.35957227146895e-10 -2645.88912164272 -3009.79647362736;-0.00096 -3.1775114179321e-10 -2577.13794148365 -3068.87068206677;-0.0009 -2.99382489084017e-10 -2507.06824993368 -3126.37479955903;-0.00084 -2.80860666761456e-10 -2435.71589594175 -3182.27940593507;-0.00078 -2.62195150932071e-10 -2363.11738469061 -3236.55589936526;-0.00072 -2.4339549121866e-10 -2289.30985892006 -3289.17651099267;-0.00066 -2.24471305874511e-10 -2214.33107992411 -3340.11431914006;-0.0006 -2.05432276862523e-10 -2138.21940823154 -3389.34326308356;-0.00054 -1.8628814490174e-10 -2061.01378397997 -3436.8381563858;-0.00048 -1.67048704483816e-10 -1982.75370699335 -3482.57469978177;-0.00042 -1.47723798861973e-10 -1903.47921657316 -3526.52949361075;-0.00036 -1.28323315015011e-10 -1823.23087101352 -3568.68004978802;-0.0003 -1.08857178588944e-10 -1742.04972685084 -3609.0048033102;-0.00024 -8.93353488188624e-11 -1659.97731785852 -3647.48312328827;-0.00018 -6.97678134335972e-11 -1577.05563379753 -3684.09532350272;-0.00012 -5.01645835458185e-11 -1493.32709893366 -3718.82267247541;-6e-05 -3.05356885301628e-11 -1408.83455033245 -3751.64740305292]  x4=[-0.0018 1.35415714894825e-09 -6688.16781747925 -1917.33848364087;-0.00174 1.3394330955528e-09 -6643.09078975579 -2068.11838030126;-0.00168 1.32402376343579e-09 -6594.61503403408 -2217.84018938386;-0.00162 1.30793703629625e-09 -6542.76535140649 -2366.42731044459;-0.00156 1.29118114440105e-09 -6487.56826912871 -2513.80372356675;-0.0015 1.27376466037409e-09 -6429.05202704797 -2659.89402825418;-0.00144 1.25569649481042e-09 -6367.24656315497 -2804.62348200757;-0.00138 1.2369858917174e-09 -6302.18349826707 -2947.91803856408;-0.00132 1.21764242378531e-09 -6233.89611985049 -3089.70438578079;-0.00126 1.19767598748976e-09 -6162.41936498985 -3229.90998314257;-0.0012 1.1770967980285e-09 -6087.78980251365 -3368.4630988751;-0.00114 1.15591538409513e-09 -6010.04561428507 -3505.2928466442;-0.00108 1.13414258249239e-09 -5929.22657566735 -3640.32922182259;-0.00102 1.1117895325879e-09 -5845.374035174 -3773.50313730555;-0.00096 1.08886767061503e-09 -5758.53089331417 -3904.74645885714;-0.0009 1.06538872382192e-09 -5668.7415806439 -4033.99203996896;-0.00084 1.04136470447158e-09 -5576.05203503467 -4161.17375621354;-0.00078 1.01680790369622e-09 -5480.50967817072 -4286.22653907478;-0.00072 9.9173088520888e-10 -5382.16339128724 -4409.08640923827;-0.00066 9.66146478875588e-10 -5281.06349016184 -4529.69050932424;-0.0006 9.4006777415137e-10 -5177.26169937204 -4647.97713604659;-0.00054 9.1350811338344e-10 -5070.81112583204 -4763.8857717814;-0.00048 8.86481084985015e-10 -4961.76623162225 -4877.35711552887;-0.00042 8.59000516483224e-10 -4850.18280612546 -4988.33311325284;-0.00036 8.31080467444695e-10 -4736.11793748399 -5096.75698758227;-0.0003 8.0273522228242e-10 -4619.6299833923 -5202.57326685962;-0.00024 7.73979282947585e-10 -4500.77854124016 -5305.72781352114;-0.00018 7.448273615101e-10 -4379.62441762149 -5406.16785179468;-0.00012 7.1529437263164e-10 -4256.22959722462 -5503.84199470075;-6e-05 6.85395425935021e-10 -4130.65721111972 -5598.70027034302]  x5=0.0017531788576868  V1=[1.492e-21 4.488e-11 4.488e-11;377 377 377;2.889 -1.992 2.721]  V2=[1.003e-22 1.265e-11 1.265e-11;377 377 377;0.8549 1.122 -0.4483]  I1=[2.499e-24 5.251e-13 5.251e-13;377 377 377;-2.215 -0.7076 -2.278]  I2=[3.136e-24 5.274e-13 5.274e-13;377 377 377;1.561 2.663 1.092]  nHarmo=1  Measurements=None  Decoupling=off  VsMag0=0  VrMag0=0  VsAngle0=0  VrAngle0=0  IsMag0=0  IrMag0=0  IsAngle0=0  IrAngle0=0
      settings: LibrarySourceBlock=sps_lib/Power Grid Elements/Distributed Parameters Line
  MPP1_3700MVA 17KV : spsSynchronousMachinepuStandardLib/Synchronous Machine pu Standard  PresetModel=No  MechanicalLoad=Mechanical power Pm  ShowDetailedParameters=on  RotorType=Salient-pole  Units=per unit standard parameters  MeasurementBus=off  NominalParameters=[3700e6 17000 60]  Reactances1=[ 1.81, 0.3, 0.23, 1.76, 0.65, 0.25, 0.15 ]  Reactances2=[ 1.305, 0.296, 0.252, 0.474, 0.243, 0.18 ]  dAxisTimeConstants=Short-circuit  qAxisTimeConstants=Open-circuit  TimeConstants1="[ 4.4849  0.0681  0.1  ]"  TimeConstants2=[ 8.0, 0.03, 1.0, 0.07 ]  TimeConstants3="[  4.49  0.0681  0.0513  ]"  TimeConstants4=[ 8.0, 0.03, 0.3371, 0.0295 ]  TimeConstants5=[ 1.01, 0.053, 0.1 ]  TimeConstants6=[ 1.3201, 0.023, 1.0, 0.07 ]  TimeConstants7=[0.012 0.003 0.003]  TimeConstants8=[ 1.3201, 0.0231, 0.3371, 0.0295 ]  StatorResistance=2.8544e-3  Mechanical=[3.5 0 32]  PolePairs=20  InitialConditions=[0 -81.9543 0.907703 0.907703 0.907703 -8.76021 -128.76 111.24 1.25655]  SetSaturation=off  Saturation=[0.6404,0.7127,0.8441,0.9214,0.9956,1.082,1.19,1.316,1.457;0.7,0.7698,0.8872,0.9466,0.9969,1.046,1.1,1.151,1.201]  LoadFlowParameters=[1,0,0,0,0]  TsPowergui=0  TsBlock=-1  IterativeModel=Trapezoidal non iterative  IterativeDiscreteModel=Trapezoidal non iterative  BusType=PV  Pref=3000e6  Qref=0  Qmin=-inf  Qmax=inf  PLF=0  QLF=0
  MPP2_500MVA 17KV : spsSynchronousMachinepuStandardLib/Synchronous Machine pu Standard  PresetModel=No  MechanicalLoad=Mechanical power Pm  ShowDetailedParameters=on  RotorType=Salient-pole  Units=per unit standard parameters  MeasurementBus=off  NominalParameters=[500e6 17000 60]  Reactances1=[ 1.81, 0.3, 0.23, 1.76, 0.65, 0.25, 0.15 ]  Reactances2=[ 1.305, 0.296, 0.252, 0.474, 0.243, 0.18 ]  dAxisTimeConstants=Short-circuit  qAxisTimeConstants=Open-circuit  TimeConstants1="[ 4.4849  0.0681  0.1  ]"  TimeConstants2=[ 8.0, 0.03, 1.0, 0.07 ]  TimeConstants3="[  4.49  0.0681  0.0513  ]"  TimeConstants4=[ 8.0, 0.03, 0.3371, 0.0295 ]  TimeConstants5=[ 1.01, 0.053, 0.1 ]  TimeConstants6=[ 1.3201, 0.023, 1.0, 0.07 ]  TimeConstants7=[0.012 0.003 0.003]  TimeConstants8=[ 1.3201, 0.0231, 0.3371, 0.0295 ]  StatorResistance=2.8544e-3  Mechanical=[3.5 0 32]  PolePairs=20  InitialConditions=[0 -81.9543 0.907703 0.907703 0.907703 -8.76021 -128.76 111.24 1.25655]  SetSaturation=off  Saturation=[0.6404,0.7127,0.8441,0.9214,0.9956,1.082,1.19,1.316,1.457;0.7,0.7698,0.8872,0.9466,0.9969,1.046,1.1,1.151,1.201]  LoadFlowParameters=[1,0,0,0,0]  TsPowergui=0  TsBlock=-1  IterativeModel=Trapezoidal non iterative  IterativeDiscreteModel=Trapezoidal non iterative  BusType=PV  Pref=400e6  Qref=0  Qmin=-inf  Qmax=inf  PLF=0  QLF=0
  MPP3-TEST2 111 km : spsDistributedParametersLineLib/Distributed Parameters Line  Phases=3  Length=111  Frequency=60  Resistance=[0.01273 0.3864]/6  Inductance="[0.9337e-3  4.1264e-3]/6"  Capacitance=[12.74e-9 7.751e-9]*6  x1=[-0.00066 -2.32339546441734e-08 0 0;-0.0006 -2.29052946552804e-08 0 0;-0.00054 -2.25649158944004e-08 0 0;-0.00048 -2.22129925055973e-08 0 0;-0.00042 -2.18497045393793e-08 -3198.25853932372 -156777.142318914;-0.00036 -2.14752378605829e-08 348.468562110914 -156809.398386032;-0.0003 -2.10897840532802e-08 3895.01738059022 -156761.427867431;-0.00024 -2.06935403227615e-08 7439.57343620596 -156633.255305716;-0.00018 -2.0286709394641e-08 10980.3232685842 -156424.946276336;-0.00012 -1.98694994111389e-08 14515.4553646852 -156136.60735404;-6e-05 -1.94421238245919e-08 18043.1610856069 -155768.386058349]  x2=[-0.00066 -1.98631434663207e-09 0 0;-0.0006 -1.55304237244361e-09 0 0;-0.00054 -1.11897583308049e-09 0 0;-0.00048 -6.84336805004866e-10 0 0;-0.00042 -2.49347657574712e-10 -8590.70930109991 -159784.744868646;-0.00036 1.85769060724472e-10 -4974.57793613612 -159938.195919491;-0.0003 6.20790736139571e-10 -1355.90148518057 -160009.819633986;-0.00024 1.05549480354317e-09 2263.46867002897 -159999.579368115;-0.00018 1.48965886030197e-09 5881.68079284284 -159907.480360987;-0.00012 1.92306078006211e-09 9496.88373908212 -159733.569732156;-6e-05 2.3554788263931e-09 13107.2279041183 -159477.936457512]  x3=[-0.00066 -1.87139100803517e-10 0 0;-0.0006 -1.68749423750628e-10 0 0;-0.00054 -1.50273411374416e-10 0 0;-0.00048 -1.31720516344212e-10 0 0;-0.00042 -1.13100230663932e-10 -812.594340459393 -2644.86803939727;-0.00036 -9.4422080815791e-11 -752.566055927189 -2662.57084836828;-0.0003 -7.56956228863856e-11 -692.152744694951 -2678.91143689461;-0.00024 -5.69304376776173e-11 -631.385315329014 -2693.88144482923;-0.00018 -3.81361258049796e-11 -570.294857569096 -2707.47321323948;-0.00012 -1.93223027857054e-11 -508.912626422208 -2719.67978832548;-6e-05 -4.98594119291001e-13 -447.270026172019 -2730.49492497786]  x4=[-0.00066 -4.84867857569848e-11 0 0;-0.0006 -6.13543475446416e-11 0 0;-0.00054 -7.41905193143966e-11 0 0;-0.00048 -8.69887338435871e-11 0 0;-0.00042 -9.97424433291762e-11 46.482628468227 -4324.85827206751;-0.00036 -1.1244512273773e-10 144.288279002278 -4322.70120116764;-0.0003 -1.25090273143744e-10 242.02010898665 -4318.33255645891;-0.00024 -1.37671425054615e-10 339.628117011248 -4311.75457302068;-0.00018 -1.50182141720552e-10 437.062365015576 -4302.97061627084;-0.00012 -1.62616022427739e-10 534.273003837979 -4291.98518024396;-6e-05 -1.74966705773053e-10 631.210298719388 -4278.80388529209]  x5=0.000627751139365274  V1=[1.134e-27 1.175e-15 1.175e-15;377 377 377;0.8883 -1.731 2.981]  V2=[1.245e-23 7.93e-13 7.93e-13;377 377 377;-1.459 -1.742 2.971]  I1=[6.861e-26 2.027e-14 2.027e-14;377 377 377;-2.79 3.007 1.436]  I2=[6.467e-26 2.017e-14 2.017e-14;377 377 377;0.1116 -0.2797 -1.851]  nHarmo=1  Measurements=None  Decoupling=off  VsMag0=0  VrMag0=0  VsAngle0=0  VrAngle0=0  IsMag0=0  IrMag0=0  IsAngle0=0  IrAngle0=0
      settings: LibrarySourceBlock=sps_lib/Power Grid Elements/Distributed Parameters Line
  MPP3_800MVA 17KV : spsSynchronousMachinepuStandardLib/Synchronous Machine pu Standard  PresetModel=No  MechanicalLoad=Mechanical power Pm  ShowDetailedParameters=on  RotorType=Salient-pole  Units=per unit standard parameters  MeasurementBus=off  NominalParameters=[800e6 17000 60]  Reactances1=[ 1.81, 0.3, 0.23, 1.76, 0.65, 0.25, 0.15 ]  Reactances2=[ 1.305, 0.296, 0.252, 0.474, 0.243, 0.18 ]  dAxisTimeConstants=Short-circuit  qAxisTimeConstants=Open-circuit  TimeConstants1="[ 4.4849  0.0681  0.1  ]"  TimeConstants2=[ 8.0, 0.03, 1.0, 0.07 ]  TimeConstants3="[  4.49  0.0681  0.0513  ]"  TimeConstants4=[ 8.0, 0.03, 0.3371, 0.0295 ]  TimeConstants5=[ 1.01, 0.053, 0.1 ]  TimeConstants6=[ 1.3201, 0.023, 1.0, 0.07 ]  TimeConstants7=[0.012 0.003 0.003]  TimeConstants8=[ 1.3201, 0.0231, 0.3371, 0.0295 ]  StatorResistance=2.8544e-3  Mechanical=[3.5 0 32]  PolePairs=20  InitialConditions=[0 -81.9543 0.907703 0.907703 0.907703 -8.76021 -128.76 111.24 1.25655]  SetSaturation=off  Saturation=[0.6404,0.7127,0.8441,0.9214,0.9956,1.082,1.19,1.316,1.457;0.7,0.7698,0.8872,0.9466,0.9969,1.046,1.1,1.151,1.201]  LoadFlowParameters=[1,0,0,0,0]  TsPowergui=0  TsBlock=-1  IterativeModel=Trapezoidal non iterative  IterativeDiscreteModel=Trapezoidal non iterative  BusType=PV  Pref=699.2e6  Qref=0  Qmin=-inf  Qmax=inf  PLF=0  QLF=0
  MPP4-TEST2 96 km : spsDistributedParametersLineLib/Distributed Parameters Line  Phases=3  Length=96  Frequency=60  Resistance=[0.01273 0.3864]/6  Inductance="[0.9337e-3  4.1264e-3]/6"  Capacitance=[12.74e-9 7.751e-9]*6  x1=[-0.0006 4.82556646649141e-09 4413.17773230548 -142505.573409162;-0.00054 5.79340907971972e-09 7635.17081699601 -142369.326497378;-0.00048 6.75828767781296e-09 10853.2576072148 -142160.240807476;-0.00042 7.71970861105143e-09 14065.7916702967 -141878.423311558;-0.00036 8.67717999872067e-09 17271.129414454 -141524.018192662;-0.0003 9.63021198076672e-09 20467.6309296692 -141097.206770995;-0.00024 1.05783169684175e-08 23653.6608267024 -140598.207411167;-0.00018 1.15210098936425e-08 26827.5890737872 -140027.275410472;-0.00012 1.24578084573221e-08 29987.7918305851 -139384.70286827;-6e-05 1.33882333760011e-08 33132.6522789717 -138670.818536547]  x2=[-0.0006 -1.55304237244361e-09 -19405.3442724175 -158834.421841427;-0.00054 -1.11897583308049e-09 -15807.9387032012 -159232.716615686;-0.00048 -6.84336805004867e-10 -12202.4455004472 -159549.544989843;-0.00042 -2.49347657574712e-10 -8590.70930109991 -159784.744868646;-0.00036 1.85769060724472e-10 -4974.57793613612 -159938.195919491;-0.0003 6.20790736139571e-10 -1355.90148518057 -160009.819633986;-0.00024 1.05549480354317e-09 2263.46867002897 -159999.579368115;-0.00018 1.48965886030197e-09 5881.68079284284 -159907.480360987;-0.00012 1.92306078006211e-09 9496.88373908212 -159733.569732156;-6e-05 2.3554788263931e-09 13107.2279041183 -159477.936457512]  x3=[-0.0006 8.25575865023996e-10 -3148.30337824027 966.935315206181;-0.00054 8.22850383828971e-10 -3169.36731342127 895.480774633023;-0.00048 8.19703917173052e-10 -3188.80974172155 823.56808954898;-0.00042 8.16138074846721e-10 -3206.62071603554 751.234051812535;-0.00036 8.121546812008e-10 -3222.79112393966 678.515668853973;-0.0003 8.07755774213084e-10 -3237.31269235445 605.450144741698;-0.00024 8.02943604445669e-10 -3250.17799177716 532.074861147941;-0.00018 7.97720633893529e-10 -3261.3804400829 458.427358223607;-0.00012 7.92089534724906e-10 -3270.9143058921 384.545315392043;-6e-05 7.86053187914186e-10 -3278.77471150287 310.466532071543]  x4=[-0.0006 -8.50701029711165e-10 2400.73149549833 -7602.27202706514;-0.00054 -8.36802361733387e-10 2572.06159585315 -7546.02939872663;-0.00048 -8.22475570205017e-10 2742.0757819693 -7485.92608231315;-0.00042 -8.07727984977329e-10 2910.68707144766 -7421.99282779195;-0.00036 -7.92567151187429e-10 3077.80919963696 -7354.26234459739;-0.0003 -7.77000825398024e-10 3243.35666376834 -7282.76928489619;-0.00024 -7.61036971629022e-10 3407.2447667002 -7207.55022585873;-0.00018 -7.44683757282988e-10 3569.38966025077 -7128.64365094551;-0.00012 -7.27949548966554e-10 3729.70838809643 -7046.08993021828;-6e-05 -7.10842908209907e-10 3888.11892821364 -6959.93129968597]  x5=0.000542919904315913  V1=[8.106e-27 2.861e-16 2.861e-16;377 377 377;-1.836 -1.712 3.001]  V2=[1.245e-23 7.93e-13 7.93e-13;377 377 377;-1.427 -1.722 2.99]  I1=[7.942e-26 2.345e-14 2.345e-14;377 377 377;-2.756 3.026 1.455]  I2=[7.544e-26 2.335e-14 2.335e-14;377 377 377;0.1775 -0.2404 -1.811]  nHarmo=1  Measurements=None  Decoupling=off  VsMag0=0  VrMag0=0  VsAngle0=0  VrAngle0=0  IsMag0=0  IrMag0=0  IsAngle0=0  IrAngle0=0
      settings: LibrarySourceBlock=sps_lib/Power Grid Elements/Distributed Parameters Line
  MPP4_3800MVA 17KV : spsSynchronousMachinepuStandardLib/Synchronous Machine pu Standard  PresetModel=No  MechanicalLoad=Mechanical power Pm  ShowDetailedParameters=on  RotorType=Salient-pole  Units=per unit standard parameters  MeasurementBus=off  NominalParameters=[3800e6 17000 60]  Reactances1=[ 1.81, 0.3, 0.23, 1.76, 0.65, 0.25, 0.15 ]  Reactances2=[ 1.305, 0.296, 0.252, 0.474, 0.243, 0.18 ]  dAxisTimeConstants=Short-circuit  qAxisTimeConstants=Open-circuit  TimeConstants1="[ 4.4849  0.0681  0.1  ]"  TimeConstants2=[ 8.0, 0.03, 1.0, 0.07 ]  TimeConstants3="[  4.49  0.0681  0.0513  ]"  TimeConstants4=[ 8.0, 0.03, 0.3371, 0.0295 ]  TimeConstants5=[ 1.01, 0.053, 0.1 ]  TimeConstants6=[ 1.3201, 0.023, 1.0, 0.07 ]  TimeConstants7=[0.012 0.003 0.003]  TimeConstants8=[ 1.3201, 0.0231, 0.3371, 0.0295 ]  StatorResistance=2.8544e-3  Mechanical=[3.5 0 32]  PolePairs=20  InitialConditions=[0 -81.9543 0.907703 0.907703 0.907703 -8.76021 -128.76 111.24 1.25655]  SetSaturation=off  Saturation=[0.6404,0.7127,0.8441,0.9214,0.9956,1.082,1.19,1.316,1.457;0.7,0.7698,0.8872,0.9466,0.9969,1.046,1.1,1.151,1.201]  LoadFlowParameters=[1,0,0,0,0]  TsPowergui=0  TsBlock=-1  IterativeModel=Trapezoidal non iterative  IterativeDiscreteModel=Trapezoidal non iterative  BusType=PV  Pref=3200e6  Qref=0  Qmin=-inf  Qmax=inf  PLF=0  QLF=0
  MPP5_4200MVA 17KV : spsSynchronousMachinepuStandardLib/Synchronous Machine pu Standard  PresetModel=No  MechanicalLoad=Mechanical power Pm  ShowDetailedParameters=on  RotorType=Salient-pole  Units=per unit standard parameters  MeasurementBus=off  NominalParameters=[4200e6 17000 60]  Reactances1=[ 1.81, 0.3, 0.23, 1.76, 0.65, 0.25, 0.15 ]  Reactances2=[ 1.305, 0.296, 0.252, 0.474, 0.243, 0.18 ]  dAxisTimeConstants=Short-circuit  qAxisTimeConstants=Open-circuit  TimeConstants1="[ 4.4849  0.0681  0.1  ]"  TimeConstants2=[ 8.0, 0.03, 1.0, 0.07 ]  TimeConstants3="[  4.49  0.0681  0.0513  ]"  TimeConstants4=[ 8.0, 0.03, 0.3371, 0.0295 ]  TimeConstants5=[ 1.01, 0.053, 0.1 ]  TimeConstants6=[ 1.3201, 0.023, 1.0, 0.07 ]  TimeConstants7=[0.012 0.003 0.003]  TimeConstants8=[ 1.3201, 0.0231, 0.3371, 0.0295 ]  StatorResistance=2.8544e-3  Mechanical=[3.5 0 32]  PolePairs=20  InitialConditions=[0 -81.9543 0.907703 0.907703 0.907703 -8.76021 -128.76 111.24 1.25655]  SetSaturation=off  Saturation=[0.6404,0.7127,0.8441,0.9214,0.9956,1.082,1.19,1.316,1.457;0.7,0.7698,0.8872,0.9466,0.9969,1.046,1.1,1.151,1.201]  LoadFlowParameters=[1,0,0,0,0]  TsPowergui=0  TsBlock=-1  IterativeModel=Trapezoidal non iterative  IterativeDiscreteModel=Trapezoidal non iterative  BusType=PV  Pref=3700e6  Qref=0  Qmin=-inf  Qmax=inf  PLF=0  QLF=0
  MPP6-CSG 186 km : spsDistributedParametersLineLib/Distributed Parameters Line  Phases=3  Length=186  Frequency=60  Resistance=[0.01273 0.3864]/6  Inductance="[0.9337e-3  4.1264e-3]/6"  Capacitance=[12.74e-9 7.751e-9]*6  x1=[-0.00108 5.1946139630209e-09 0 0;-0.00102 6.18626199143655e-09 0 0;-0.00096 7.1747450139084e-09 0 0;-0.0009 8.15955730425709e-09 0 0;-0.00084 9.14019501431765e-09 0 0;-0.00078 1.01161564317175e-08 0 0;-0.00072 1.10869422365618e-08 0 0;-0.00066 1.20520557568947e-08 -124252.084908224 -195825.649274526;-0.0006 1.3011003222806e-08 -119791.202249251 -198585.862180897;-0.00054 1.39632940190529e-08 -115269.03219772 -201244.474890732;-0.00048 1.49084409360676e-08 -110687.88837939 -203800.127208643;-0.00042 1.5845960419223e-08 -106050.114592089 -206251.51161568;-0.00036 1.67753728162283e-08 -101358.083606581 -208597.373938285;-0.0003 1.76962026225276e-08 -96614.1959526178 -210836.513989947;-0.00024 1.8607978724577e-08 -91820.8786907803 -212967.78618524;-0.00018 1.9510234640875e-08 -86980.5841707498 -214990.100125929;-0.00012 2.0402508760623e-08 -82095.7887766411 -216902.421158834;-6e-05 2.1284344579894e-08 -77168.9916600386 -218703.770905177]  x2=[-0.00108 -6.5450703365461e-09 0 0;-0.00102 -5.13480871258508e-09 0 0;-0.00096 -3.72192002560633e-09 0 0;-0.0009 -2.30712713556932e-09 0 0;-0.00084 -8.91153876658933e-10 0 0;-0.00078 5.25275313041382e-10 0 0;-0.00072 1.94143576218557e-09 0 0;-0.00066 3.35660293692021e-09 -135536.539986396 -206838.589363699;-0.0006 4.77005281156944e-09 -130823.684571695 -209851.213359525;-0.00054 6.18106223905983e-09 -126043.897342623 -212756.473596992;-0.00048 7.58890932089581e-09 -121199.623726648 -215552.883691278;-0.00042 8.9928737764963e-09 -116293.342143662 -218239.012947309;-0.00036 1.03922373117035e-08 -111327.562737982 -220813.487091723;-0.0003 1.17862839862756e-08 -106304.826094108 -223274.988975977;-0.00024 1.31743005801749e-08 -101227.701936917 -225622.259250223;-0.00018 1.45555769584642e-08 -96098.7878169425 -227854.097007616;-0.00012 1.59294064346254e-08 -90920.7077814192 -229969.360398721;-6e-05 1.72950861321131e-08 -85696.1110317734 -231966.967215701]  x3=[-0.00108 -4.33960329995218e-10 0 0;-0.00102 -4.29237509486254e-10 0 0;-0.00096 -4.2429508313604e-10 0 0;-0.0009 -4.19135579581222e-10 0 0;-0.00084 -4.13761638519155e-10 0 0;-0.00078 -4.08176009357385e-10 0 0;-0.00072 -4.02381549807003e-10 0 0;-0.00066 -3.96381224420583e-10 -4311.32725878193 -2976.24262676765;-0.0006 -3.90178103075467e-10 -4242.90877753926 -3072.99351045316;-0.00054 -3.83775359403155e-10 -4172.31954576606 -3168.17219387633;-0.00048 -3.7717626916562e-10 -4099.59567821765 -3261.72998186402;-0.00042 -3.70384208579362e-10 -4024.77438176844 -3353.61900852315;-0.00036 -3.63402652588083e-10 -3947.89393637624 -3443.79226172976;-0.0003 -3.5623517308483e-10 -3868.9936754975 -3532.20360718131;-0.00024 -3.48885437084558e-10 -3788.11396596359 -3618.80781199981;-0.00018 -3.41357204848012e-10 -3705.29618732839 -3703.56056787381;-0.00012 -3.3365432795791e-10 -3620.58271069776 -3786.41851372735;-6e-05 -3.25780747348402e-10 -3534.01687705165 -3867.3392579043]  x4=[-0.00108 2.5725909149359e-10 0 0;-0.00102 2.70898161456022e-10 0 0;-0.00096 2.8439863491343e-10 0 0;-0.0009 2.97753604774134e-10 0 0;-0.00084 3.10956238388782e-10 0 0;-0.00078 3.2399978104606e-10 0 0;-0.00072 3.36877559428526e-10 0 0;-0.00066 3.49582985026808e-10 -2488.30022743085 -5192.86541117799;-0.0006 3.62109557510399e-10 -2370.21384439297 -5247.81699437593;-0.00054 3.74450868053352e-10 -2250.91481615579 -5300.08369743104;-0.00048 3.86600602613153e-10 -2130.46417830653 -5349.63877973226;-0.00042 3.98552545161099e-10 -2008.92355561721 -5396.45688798381;-0.00036 4.10300580862536e-10 -1886.35513051619 -5440.5140691764;-0.0003 4.21838699205321e-10 -1762.82161127456 -5481.78778284207;-0.00024 4.3316099707491e-10 -1638.38619992341 -5520.25691258624;-0.00018 4.442616817745e-10 -1513.11255991848 -5555.90177689131;-0.00012 4.55135073988682e-10 -1387.06478356879 -5588.70413918607;-6e-05 4.65775610689082e-10 -1260.30735924581 -5618.64721717583]  x5=0.00105190731461208  V1=[8.574e-27 4.511e-17 4.511e-17;377 377 377;-2.265 1.301 -0.2697]  V2=[1.073e-22 6.76e-12 6.76e-12;377 377 377;0.1921 1.269 -0.3021]  I1=[3.519e-25 1.037e-13 1.037e-13;377 377 377;-1.143 -0.2664 -1.837]  I2=[3.187e-25 1.028e-13 1.028e-13;377 377 377;1.591 2.633 1.062]  nHarmo=1  Measurements=None  Decoupling=off  VsMag0=0  VrMag0=0  VsAngle0=0  VrAngle0=0  IsMag0=0  IrMag0=0  IsAngle0=0  IrAngle0=0
      settings: LibrarySourceBlock=sps_lib/Power Grid Elements/Distributed Parameters Line
  MPP6_490MVA 17KV : spsSynchronousMachinepuStandardLib/Synchronous Machine pu Standard  PresetModel=No  MechanicalLoad=Mechanical power Pm  ShowDetailedParameters=on  RotorType=Salient-pole  Units=per unit standard parameters  MeasurementBus=off  NominalParameters=[490e6 13800 60]  Reactances1=[ 1.81, 0.3, 0.23, 1.76, 0.65, 0.25, 0.15 ]  Reactances2=[ 1.305, 0.296, 0.252, 0.474, 0.243, 0.18 ]  dAxisTimeConstants=Short-circuit  qAxisTimeConstants=Open-circuit  TimeConstants1="[ 4.4849  0.0681  0.1  ]"  TimeConstants2=[ 8.0, 0.03, 1.0, 0.07 ]  TimeConstants3="[  4.49  0.0681  0.0513  ]"  TimeConstants4=[ 8.0, 0.03, 0.3371, 0.0295 ]  TimeConstants5=[ 1.01, 0.053, 0.1 ]  TimeConstants6=[ 1.3201, 0.023, 1.0, 0.07 ]  TimeConstants7=[0.012 0.003 0.003]  TimeConstants8=[ 1.3201, 0.0231, 0.3371, 0.0295 ]  StatorResistance=2.8544e-3  Mechanical=[3.5 0 32]  PolePairs=20  InitialConditions=[0 -81.9543 0.907703 0.907703 0.907703 -8.76021 -128.76 111.24 1.25655]  SetSaturation=off  Saturation=[0.6404,0.7127,0.8441,0.9214,0.9956,1.082,1.19,1.316,1.457;0.7,0.7698,0.8872,0.9466,0.9969,1.046,1.1,1.151,1.201]  LoadFlowParameters=[1,0,0,0,0]  TsPowergui=0  TsBlock=-1  IterativeModel=Trapezoidal non iterative  IterativeDiscreteModel=Trapezoidal non iterative  BusType=PV  Pref=415e6  Qref=0  Qmin=-inf  Qmax=inf  PLF=0  QLF=0
  PNS-CON 260 km : spsDistributedParametersLineLib/Distributed Parameters Line  Phases=3  Length=271  Frequency=60  Resistance=[0.01273 0.3864]/6  Inductance="[0.9337e-3  4.1264e-3]/6"  Capacitance=[12.74e-9 7.751e-9]*6  x1=[-0.00156 2.84165066463403e-08 -185077.136849389 -161589.337578389;-0.0015 2.96847671959942e-08 -181375.025022969 -165734.020683138;-0.00144 3.09378404702392e-08 -177580.118382323 -169793.911200493;-0.00138 3.21750853736341e-08 -173694.358471809 -173766.932015447;-0.00132 3.33958689088247e-08 -169719.733317998 -177651.050457138;-0.00126 3.45995665003967e-08 -165658.276412561 -181444.279338801;-0.0012 3.57855623144207e-08 -161512.065671899 -185144.67797445;-0.00114 3.69532495735235e-08 -157283.222374039 -188750.353171767;-0.00108 3.81020308673269e-08 -152973.910073352 -192259.460200695;-0.00102 3.9231318458094e-08 -148586.33349364 -195670.203737238;-0.00096 4.03405345814265e-08 -144122.737400152 -198980.83878198;-0.0009 4.14291117418598e-08 -139585.405451128 -202189.671552858;-0.00084 4.24964930032039e-08 -134976.659029434 -205295.060351734;-0.00078 4.35421322734828e-08 -130298.856054899 -208295.416404317;-0.00072 4.45654945843244e-08 -125554.389777959 -211189.204673011;-0.00066 4.5566056364661e-08 -120745.687555231 -213974.944642267;-0.0006 4.65433057085976e-08 -115875.209607626 -216651.211076041;-0.00054 4.74967426373122e-08 -110945.447761658 -219216.634746975;-0.00048 4.84258793548547e-08 -105958.924174579 -221669.903136914;-0.00042 4.93302404977119e-08 -100918.190043996 -224009.76110842;-0.00036 5.02093633780124e-08 -95825.8243026334 -226235.011546918;-0.0003 5.10627982202463e-08 -90684.4322988997 -228344.515973166;-0.00024 5.18901083913787e-08 -85496.6444639462 -230337.195125721;-0.00018 5.26908706242392e-08 -80265.1149658885 -232212.029513108;-0.00012 5.34646752340729e-08 -74992.5203518856 -233968.05993541;-6e-05 5.42111263281433e-08 -69681.5581787681 -235604.387975017]  x2=[-0.00156 1.25267881990069e-09 -228427.246404569 -181790.086778468;-0.0015 3.34335418282189e-09 -224257.151076829 -186910.078287832;-0.00144 5.43231902396511e-09 -219972.321646802 -191934.443147443;-0.00138 7.51850459031793e-09 -215574.9503124 -196860.6107994;-0.00132 9.60084355079635e-09 -211067.28685005 -201686.060925305;-0.00126 1.1678270542311e-08 -206451.637463673 -206408.324735711;-0.0012 1.37497227148266e-08 -201730.363604783 -211024.986233195;-0.00114 1.58141402751356e-08 -196905.880764323 -215533.683448429;-0.00108 1.78704670290681e-08 -191980.657236862 -219932.109648606;-0.00102 1.99176509218603e-08 -186957.212857764 -224218.014517609;-0.00096 2.1954644576405e-08 -181838.117713996 -228389.205307311;-0.0009 2.39804058291092e-08 -176625.990829223 -232443.547959432;-0.00084 2.59938982630843e-08 -171323.498823869 -236378.968197353;-0.00078 2.7994091738396e-08 -165933.354550822 -240193.452587363;-0.00072 2.9979962919103e-08 -160458.315707492 -243885.049568766;-0.00066 3.19504957968145e-08 -154901.183424916 -247451.870452331;-0.0006 3.39046822104992e-08 -149264.800834656 -250892.090386587;-0.00054 3.58415223622784e-08 -143552.051614192 -254203.94929145;-0.00048 3.77600253289419e-08 -137765.858511586 -257385.752758705;-0.00042 3.9659209568922e-08 -131909.181850144 -260435.872918908;-0.00036 4.15381034244688e-08 -125985.018013867 -263352.749274224;-0.0003 4.33957456187677e-08 -119996.397914438 -266134.889496811;-0.00024 4.52311857477469e-08 -113946.385440558 -268780.870192325;-0.00018 4.70434847663213e-08 -107838.075890399 -271289.337628149;-0.00012 4.88317154688256e-08 -101674.594387996 -273659.008425992;-6e-05 5.05949629633897e-08 -95459.0942843738 -275888.670218487]  x3=[-0.00156 -4.78670398384426e-10 -6080.74420272706 -103.915055482171;-0.0015 -4.7336383362794e-10 -6076.83774798028 -241.420359255611;-0.00144 -4.67815087187412e-10 -6069.82227075458 -378.802147912322;-0.00138 -4.6202699790405e-10 -6059.70136029774 -515.990134390701;-0.00132 -4.56002527071282e-10 -6046.48019465457 -652.914130781925;-0.00126 -4.49744756919707e-10 -6030.1655380177 -789.504084239374;-0.0012 -4.43256889040165e-10 -6010.76573726694 -925.690112818969;-0.00114 -4.36542242745744e-10 -5988.29071769881 -1061.40254123206;-0.00108 -4.29604253373561e-10 -5962.75197794861 -1196.57193649259;-0.00102 -4.22446470527178e-10 -5934.16258410751 -1331.1291434403;-0.00096 -4.1507255626056e-10 -5902.53716303766 -1465.0053201218;-0.0009 -4.074862832045e-10 -5867.89189488886 -1598.13197301133;-0.00084 -3.99691532636472e-10 -5830.24450482045 -1730.44099205338;-0.00078 -3.91692292494897e-10 -5789.61425393285 -1861.86468550903;-0.00072 -3.8349265533884e-10 -5746.02192941316 -1992.33581458827;-0.00066 -3.75096816254183e-10 -5699.48983390011 -2121.78762785063;-0.0006 -3.66509070707337e-10 -5650.04177407357 -2250.15389535646;-0.00054 -3.57733812347608e-10 -5597.70304847464 -2377.36894255136;-0.00048 -3.48775530759322e-10 -5542.50043456246 -2503.36768386652;-0.00042 -3.39638809164868e-10 -5484.46217501432 -2628.08565601769;-0.00036 -3.30328322079842e-10 -5423.61796327624 -2751.45905098582;-0.0003 -3.20848832921474e-10 -5359.9989283712 -2873.42474866233;-0.00024 -3.11205191571579e-10 -5293.63761897302 -2993.92034914265;-0.00018 -3.01402331895265e-10 -5224.5679867538 -3112.88420465106;-0.00012 -2.91445269216679e-10 -5152.82536901363 -3230.25545108089;-6e-05 -2.81339097753072e-10 -5078.44647060142 -3345.97403913368]  x4=[-0.00156 3.59284358612378e-10 -4342.03754850242 -5812.16703025074;-0.0015 3.803424494344e-10 -4209.46960490609 -5908.88726276532;-0.00144 4.01205950031371e-10 -4074.74801887784 -6002.58439937259;-0.00138 4.21864186250872e-10 -3937.94171647045 -6093.21050288613;-0.00132 4.42306588957534e-10 -3799.12069031611 -6180.71920731681;-0.00126 4.62522699440398e-10 -3658.35596381692 -6265.06574159447;-0.0012 4.82502174763793e-10 -3515.71955480801 -6346.20695247362;-0.00114 5.02234793058963e-10 -3371.28443871182 -6424.10132661147;-0.00108 5.21710458753772e-10 -3225.12451120262 -6498.70901180688;-0.00102 5.40919207737781e-10 -3077.31455040003 -6569.99183738951;-0.00096 5.59851212460075e-10 -2927.93017861123 -6637.91333374864;-0.0009 5.78496786957213e-10 -2777.04782364112 -6702.43875099169;-0.00084 5.96846391808751e-10 -2624.74467969048 -6763.5350767229;-0.00078 6.14890639017788e-10 -2471.09866786202 -6821.1710529331;-0.00072 6.3262029681403e-10 -2316.18839629442 -6875.31719199188;-0.00066 6.50026294376943e-10 -2160.09311994504 -6925.94579173397;-0.0006 6.67099726476548e-10 -2002.89270004156 -6973.03094963225;-0.00054 6.83831858029501e-10 -1844.66756322354 -7016.5485760499;-0.00048 7.00214128568127e-10 -1685.49866039464 -7056.47640656514;-0.00042 7.16238156620108e-10 -1525.46742530665 -7092.79401336208;-0.00036 7.31895743996603e-10 -1364.65573289647 -7125.48281568202;-0.0003 7.47178879986591e-10 -1203.1458573974 -7154.52608932968;-0.00024 7.62079745455299e-10 -1041.02043024611 -7179.90897522959;-0.00018 7.76590716844617e-10 -878.362397806857 -7201.61848702831;-0.00012 7.90704370073452e-10 -715.254978934617 -7219.64351773846;-6e-05 8.0441348433602e-10 -551.781622398761 -7233.97484542125]  x5=0.00153261764655846  V1=[1.516e-17 3.586e-06 3.586e-06;377 377 377;3.054 -1.986 2.727]  V2=[2.167e-13 0.2213 0.2213;377 377 377;-0.8435 -2.017 2.695]  I1=[4.914e-16 0.002352 0.002352;377 377 377;-2.188 2.73 1.159]  I2=[4.262e-16 0.002322 0.002322;377 377 377;0.3532 -0.7649 -2.336]  nHarmo=1  Measurements=None  Decoupling=off  VsMag0=0  VrMag0=0  VsAngle0=0  VrAngle0=0  IsMag0=0  IrMag0=0  IsAngle0=0  IrAngle0=0
      settings: LibrarySourceBlock=sps_lib/Power Grid Elements/Distributed Parameters Line
  PNS3 : spsThreePhaseVIMeasurementLib/Three-Phase V-I Measurement  VoltageMeasurement=no  SetLabelV=off  LabelV=Vabc  Vpu=off  VpuLL=off  CurrentMeasurement=no  SetLabelI=off  LabelI=Iabc  Ipu=off  Pbase=100e6  Vbase=500e3  OutputType=Complex  PhasorSimulation=off  PSBequivalent=0
  Regulators 1 : Subsystem
  Regulators 2 : Subsystem
  Regulators 3 : Subsystem
  Regulators 4 : Subsystem
  Regulators 5 : Subsystem
  Regulators 6 : Subsystem
  TEST 1 : spsThreePhaseVIMeasurementLib/Three-Phase V-I Measurement  VoltageMeasurement=no  SetLabelV=off  LabelV=Vabc  Vpu=off  VpuLL=off  CurrentMeasurement=no  SetLabelI=off  LabelI=Iabc  Ipu=off  Pbase=100e6  Vbase=500e3  OutputType=Complex  PhasorSimulation=off  PSBequivalent=0
  TEST1-MPP2 187 km : spsDistributedParametersLineLib/Distributed Parameters Line  Phases=3  Length=187  Frequency=60  Resistance=[0.01273 0.3864]/6  Inductance="[0.9337e-3  4.1264e-3]/6"  Capacitance=[12.74e-9 7.751e-9]*6  x1=[-0.00108 3.94983894749446e-08 0 0;-0.00102 3.96842925883609e-08 0 0;-0.00096 3.98498924844075e-08 0 0;-0.0009 3.99951044391178e-08 0 0;-0.00084 4.01198541593724e-08 0 0;-0.00078 4.02240778209095e-08 0 0;-0.00072 4.03077221009778e-08 0 0;-0.00066 4.03707442056183e-08 116022.210330946 180918.68670654;-0.0006 4.04131118915575e-08 120084.492979149 178248.281862339;-0.00054 4.04348034827046e-08 124085.338181837 175486.681903487;-0.00048 4.04358078812407e-08 128022.699032678 172635.299715552;-0.00042 4.04161245732969e-08 131894.561105106 169695.594118349;-0.00036 4.03757636292173e-08 135698.943482942 166669.069119581;-0.0003 4.03147456984066e-08 139433.899773864 163557.273145362;-0.00024 4.02331019987658e-08 143097.519105219 160361.79824801;-0.00018 4.01308743007202e-08 146687.927101662 157084.279291529;-0.00012 4.00081149058491e-08 150203.286844118 153726.393115179;-6e-05 3.98648866201271e-08 153641.799809587 150289.857675574]  x2=[-0.00108 5.11445802609634e-08 0 0;-0.00102 5.13697709105391e-08 0 0;-0.00096 5.15686798361128e-08 0 0;-0.0009 5.17412052722027e-08 0 0;-0.00084 5.18872589516078e-08 0 0;-0.00078 5.2006766150567e-08 0 0;-0.00072 5.2099665726989e-08 0 0;-0.00066 5.21659101517339e-08 117258.781838056 189238.873300873;-0.0006 5.220546553293e-08 121508.931138218 186538.372003897;-0.00054 5.22183116333133e-08 125696.914223982 183742.434228971;-0.00048 5.22044418805816e-08 129820.588445818 180852.490429524;-0.00042 5.21638633707567e-08 133877.844055796 177870.019154203;-0.00036 5.20965968645538e-08 137866.605286977 174796.546290423;-0.0003 5.20026767767606e-08 141784.831415412 171633.644283692;-0.00024 5.18821511586295e-08 145630.517804211 168382.931333121;-0.00018 5.17350816732937e-08 149401.69692916 165046.07056352;-0.00012 5.15615435642194e-08 153096.439385334 161624.769174518;-6e-05 5.13616256167099e-08 156712.854874221 158120.777567125]  x3=[-0.00108 3.05002109749534e-10 0 0;-0.00102 3.13015653242688e-10 0 0;-0.00096 3.2086905214378e-10 0 0;-0.0009 3.28558288508816e-10 0 0;-0.00084 3.36079428382392e-10 0 0;-0.00078 3.43428623810373e-10 0 0;-0.00072 3.50602114808582e-10 0 0;-0.00066 3.57596231286473e-10 1309.15068214794 4436.42951918252;-0.0006 3.64407394924819e-10 1409.15754436895 4405.68500271247;-0.00054 3.71032121006447e-10 1508.44345555203 4372.68645638733;-0.00048 3.77467020199082e-10 1606.95761919042 4337.45076287315;-0.00042 3.83708800289395e-10 1704.64963361767 4299.99594940181;-0.00036 3.89754267867357e-10 1801.46951779406 4260.34117854797;-0.0003 3.95600329960047e-10 1897.36773687781 4218.50673842513;-0.00024 4.01243995614076e-10 1992.29522756806 4174.51403230587;-0.00018 4.06682377425812e-10 2086.20342320649 4128.38556767153;-0.00012 4.11912693018631e-10 2179.04427862501 4080.14494469697;-6e-05 4.16932266466429e-10 2270.77029472647 4029.8168441763]  x4=[-0.00108 3.55918797222692e-10 0 0;-0.00102 3.54241274067868e-10 0 0;-0.00096 3.52382514531606e-10 0 0;-0.0009 3.50343469589628e-10 0 0;-0.00084 3.48125182455006e-10 0 0;-0.00078 3.45728788044426e-10 0 0;-0.00072 3.43155512397549e-10 0 0;-0.00066 3.40406672049744e-10 2829.05080128044 4342.16353283811;-0.0006 3.37483673358527e-10 2926.53678376312 4277.06688471235;-0.00054 3.34388011784038e-10 3022.52549595104 4209.78201013726;-0.00048 3.3112127112394e-10 3116.96782824538 4140.34333329795;-0.00042 3.27685122703118e-10 3209.81546220385 4068.78638030458;-0.00036 3.24081324518596e-10 3301.02089526129 3995.14776101652;-0.0003 3.20311720340116e-10 3390.53746503285 3919.46515031209;-0.00024 3.1637823876683e-10 3478.31937318738 3841.77726881336;-0.00018 3.12282892240593e-10 3564.32170887863 3762.12386307602;-0.00012 3.08027776016361e-10 3648.50047172253 3680.54568525428;-6e-05 3.03615067090221e-10 3730.81259430855 3597.0844722513]  x5=0.00105756273028204  V1=[5.148e-22 3.64e-12 3.64e-12;377 377 377;-2.284 2.392 -2.32]  V2=[4.457e-19 3.159e-07 3.159e-07;377 377 377;1.876 2.36 -2.352]  I1=[1.453e-21 4.823e-09 4.823e-09;377 377 377;0.5394 0.8251 2.396]  I2=[1.317e-21 4.781e-09 4.781e-09;377 377 377;-3.011 -2.56 -0.9894]  nHarmo=1  Measurements=None  Decoupling=off  VsMag0=0  VrMag0=0  VsAngle0=0  VrAngle0=0  IsMag0=0  IrMag0=0  IsAngle0=0  IrAngle0=0
      settings: LibrarySourceBlock=sps_lib/Power Grid Elements/Distributed Parameters Line
  TEST1-PNS 235 km : spsDistributedParametersLineLib/Distributed Parameters Line  Phases=3  Length=235  Frequency=60  Resistance=[0.01273 0.3864]/6  Inductance="[0.9337e-3  4.1264e-3]/6"  Capacitance=[12.74e-9 7.751e-9]*6  x1=[-0.00138 4.96289006876161e-08 -153997.917543823 -160765.384956069;-0.00132 4.99835050640778e-08 -150322.395342068 -164207.341991158;-0.00126 5.03125369557597e-08 -146569.965425218 -167565.287515881;-0.0012 5.06158280238663e-08 -142742.547605754 -170837.50354326;-0.00114 5.08932230990829e-08 -138842.100061357 -174022.315947112;-0.00108 5.11445802609634e-08 -134870.618333061 -177118.095318563;-0.00102 5.13697709105391e-08 -130830.134304303 -180123.257799684;-0.00096 5.15686798361128e-08 -126722.715161373 -183036.265893818;-0.0009 5.17412052722027e-08 -122550.462335799 -185855.6292522;-0.00084 5.18872589516078e-08 -118315.510429222 -188579.90543644;-0.00078 5.2006766150567e-08 -114020.02612129 -191207.700656502;-0.00072 5.2099665726989e-08 -109666.207061147 -193737.670483796;-0.00066 5.21659101517339e-08 -105256.280743073 -196168.52053901;-0.0006 5.220546553293e-08 -100792.503366858 -198499.007154339;-0.00054 5.22183116333133e-08 -96277.1586834895 -200727.938009768;-0.00048 5.22044418805816e-08 -91712.556826741 -202854.172743085;-0.00042 5.21638633707567e-08 -87101.0331312668 -204876.623533313;-0.00036 5.20965968645538e-08 -82444.9469378006 -206794.255657256;-0.0003 5.20026767767606e-08 -77746.6803860735 -208606.088018887;-0.00024 5.18821511586295e-08 -73008.6371960675 -210311.193651289;-0.00018 5.17350816732937e-08 -68233.2414382274 -211908.700190916;-0.00012 5.15615435642194e-08 -63422.9362932622 -213397.790323903;-6e-05 5.13616256167099e-08 -58580.1828021682 -214777.702204221]  x2=[-0.00138 3.02185083694915e-08 -206219.825689165 -194979.465858924;-0.00132 3.15976485409716e-08 -201757.102841495 -199593.807092726;-0.00126 3.29606227716006e-08 -197191.157331968 -204106.03244675;-0.0012 3.43067337385774e-08 -192524.325182676 -208513.833383128;-0.00114 3.5635292746658e-08 -187758.994031181 -212814.954789455;-0.00108 3.69456200805049e-08 -182897.601908952 -217007.196132543;-0.00102 3.82370453524421e-08 -177942.635994027 -221088.412584258;-0.00096 3.95089078454376e-08 -172896.631338526 -225056.516118851;-0.0009 4.07605568511387e-08 -167762.16957167 -228909.476581231;-0.00084 4.19913520027862e-08 -162541.877578972 -232645.322725631;-0.00078 4.32006636028382e-08 -157238.426158276 -236262.143224133;-0.00072 4.43878729451344e-08 -151854.528653326 -239758.08764454;-0.00066 4.55523726314384e-08 -146392.939565567 -243131.367397087;-0.0006 4.6693566882193e-08 -140856.453144896 -246380.256649523;-0.00054 4.78108718413328e-08 -135247.901960069 -249503.093210074;-0.00048 4.89037158749952e-08 -129570.155449504 -252498.279377851;-0.00042 4.99715398639792e-08 -123826.118453231 -255364.282760266;-0.00036 5.10137974898009e-08 -118018.729726713 -258099.637057032;-0.0003 5.20299555142002e-08 -112150.960437332 -260702.942810347;-0.00024 5.30194940519554e-08 -106225.812644279 -263172.868120884;-0.00018 5.39819068368661e-08 -100246.317762651 -265508.149329214;-0.00012 5.4916701480768e-08 -94215.5350125155 -267707.591662321;-6e-05 5.58233997254484e-08 -88136.5498537651 -269770.069844866]  x3=[-0.00138 -4.15484311962405e-10 -6569.4713460361 721.833103208731;-0.00132 -4.13488371369596e-10 -6584.116157804 573.062834998277;-0.00126 -4.11280882485607e-10 -6595.39241408508 423.999377252454;-0.0012 -4.08862974702542e-10 -6603.29434573827 274.718993590622;-0.00114 -4.062358850667e-10 -6607.81790998934 125.298058615445;-0.00108 -4.03400957645682e-10 -6608.96079249922 -24.1869811617621;-0.00102 -4.00359642840739e-10 -6606.7224085481 -173.659646432482;-0.00096 -3.97113496644724e-10 -6601.10390333457 -323.043464219226;-0.0009 -3.93664179846011e-10 -6592.10815138973 -472.262007000519;-0.00084 -3.90013457178812e-10 -6579.73975510647 -621.238931812631;-0.00078 -3.861631964203e-10 -6564.0050423849 -769.898019308053;-0.00072 -3.82115367435023e-10 -6544.91206339477 -918.163212750716;-0.00066 -3.77872041167087e-10 -6522.47058645694 -1065.95865692803;-0.0006 -3.73435388580617e-10 -6496.69209304567 -1213.20873695981;-0.00054 -3.68807679549057e-10 -6467.58977191454 -1359.83811698424;-0.00048 -3.63991281693857e-10 -6435.17851234878 -1505.7717787011;-0.00042 -3.58988659173157e-10 -6399.47489654768 -1650.93505975252;-0.00036 -3.53802371421076e-10 -6360.4971911408 -1795.25369192159;-0.0003 -3.4843507183826e-10 -6318.26533784245 -1938.65383912941;-0.00024 -3.42889506434351e-10 -6272.80094324915 -2081.06213521092;-0.00018 -3.37168512423082e-10 -6224.12726778525 -2222.40572145044;-0.00012 -3.31275016770698e-10 -6172.2692138025 -2362.61228385754;-6e-05 -3.25212034698477e-10 -6117.25331283954 -2501.61009016416]  x4=[-0.00138 8.59746923211455e-10 -2555.05455259702 -7318.19590051786;-0.00132 8.74267482932727e-10 -2388.88134795164 -7374.11382348341;-0.00126 8.88340751255125e-10 -2221.48594746719 -7426.25901355892;-0.0012 9.01959528034531e-10 -2052.95399372367 -7474.60479230159;-0.00114 9.15116845653098e-10 -1883.37171078274 -7519.12642511771;-0.00108 9.27805972584014e-10 -1712.82586007386 -7559.80113391726;-0.00102 9.40020416835473e-10 -1541.40369600559 -7596.60810876763;-0.00096 9.51753929272099e-10 -1369.19292132457 -7629.52851854038;-0.0009 9.63000506812119e-10 -1196.28164224523 -7658.54552054556;-0.00084 9.7375439549865e-10 -1022.75832337297 -7683.64426914879;-0.00078 9.84010093443532e-10 -848.711742444076 -7704.81192336649;-0.00072 9.93762353642191e-10 -674.230944905356 -7722.03765343565;-0.00066 1.00300618665811e-09 -499.405198356867 -7735.31264635445;-0.0006 1.01173686317551e-09 -324.323946880951 -7744.63011039124;-0.00054 1.01994991641897e-09 -149.076765280994 -7749.98527855924;-0.00048 1.02764114443867e-09 26.2466867467033 -7751.37541105547;-0.00042 1.03480661226026e-09 201.556710484478 -7748.79979666245;-0.00036 1.04144265389798e-09 376.763614084829 -7742.25975311211;-0.0003 1.04754587423033e-09 551.777758458423 -7731.75862641156;-0.00024 1.05311315073699e-09 726.509603135109 -7717.30178913126;-0.00018 1.05814163509645e-09 900.869752074477 -7698.8966376563;-0.00012 1.06262875464318e-09 1074.76899940252 -7676.55258840227;-6e-05 1.06657221368391e-09 1248.11837505103 -7650.28107299762]  x5=0.00132902268243999  V1=[4.457e-19 3.159e-07 3.159e-07;377 377 377;1.774 1.251 -0.3202]  V2=[2.934e-17 4.144e-06 4.144e-06;377 377 377;-1.608 -1.933 2.78]  I1=[7.734e-20 5.426e-08 5.426e-08;377 377 377;-2.952 2.797 1.226]  I2=[6.83e-20 5.366e-08 5.366e-08;377 377 377;-0.313 -0.6082 -2.179]  nHarmo=1  Measurements=None  Decoupling=off  VsMag0=0  VrMag0=0  VsAngle0=0  VrAngle0=0  IsMag0=0  IrMag0=0  IsAngle0=0  IrAngle0=0
      settings: LibrarySourceBlock=sps_lib/Power Grid Elements/Distributed Parameters Line
  TEST2 : spsThreePhaseVIMeasurementLib/Three-Phase V-I Measurement  VoltageMeasurement=no  SetLabelV=off  LabelV=Vabc  Vpu=off  VpuLL=off  CurrentMeasurement=no  SetLabelI=off  LabelI=Iabc  Ipu=off  Pbase=100e6  Vbase=500e3  OutputType=Complex  PhasorSimulation=off  PSBequivalent=0
  CON-a : PMIOPort  Side=Left
  CON-b : PMIOPort  Port=2  Side=Left
  CON-c : PMIOPort  Port=3  Side=Left
  SAT-a : PMIOPort  Port=4  Side=Left
  SAT-b : PMIOPort  Port=5  Side=Left
  SAT-c : PMIOPort  Port=6  Side=Left
  wires:
  Regulators 1/2(Vf) -> MPP1_3700MVA 17KV/2
  Regulators 1/1(Pm) -> MPP1_3700MVA 17KV/1
  Regulators 4/1(Pm) -> MPP4_3800MVA 17KV/1
  Regulators 4/2(Vf) -> MPP4_3800MVA 17KV/2
  MPP1_3700MVA 17KV/1 -> Regulators 1/1(m)
  Regulators 3/1(Pm) -> MPP3_800MVA 17KV/1
  Regulators 2/1(Pm) -> MPP2_500MVA 17KV/1
  MPP4_3800MVA 17KV/1 -> Regulators 4/1(m)
  MPP3_800MVA 17KV/1 -> Regulators 3/1(m)
  Regulators 3/2(Vf) -> MPP3_800MVA 17KV/2
  Regulators 2/2(Vf) -> MPP2_500MVA 17KV/2
  MPP2_500MVA 17KV/1 -> Regulators 2/1(m)
  Regulators 5/1(Pm) -> MPP5_4200MVA 17KV/1
  Regulators 5/2(Vf) -> MPP5_4200MVA 17KV/2
  MPP5_4200MVA 17KV/1 -> Regulators 5/1(m)
  Regulators 6/1(Pm) -> MPP6_490MVA 17KV/1
  Regulators 6/2(Vf) -> MPP6_490MVA 17KV/2
  MPP6_490MVA 17KV/1 -> Regulators 6/1(m)
  connections:
  CLP-CSG 103 km/LConn3 -- Cs CSGN/LConn3
  CLP-TEST2 288 km/RConn1 -- Cs CLPS/LConn1 -- Cs AND/RConn1
  CLP 1/LConn3 -- 4200 MVA 17KV :650KV Transformer/RConn3 -- Cs CLPN/RConn3 -- Cs CLPS/RConn3
  "500 MVA 17KV :650KV Transformer "/LConn3 -- 1980 MVar/LConn3 -- TEST1-MPP2 187 km/LConn1
  CLP-CSG 103 km/RConn1 -- 990 MVar3/LConn1 -- CLP 1/RConn1 -- Load Flow Bus7/LConn1
  MPP3-TEST2 111 km/RConn2 -- 660 MVar4/LConn2 -- MPP4-TEST2 96 km/RConn2 -- TEST2/LConn2
  MPP2_500MVA 17KV/RConn2 -- 25 MW/LConn2 -- "500 MVA 17KV :650KV Transformer "/RConn2
  TEST1-PNS 235 km/LConn2 -- TEST 1/LConn2 -- TEST1-MPP2 187 km/RConn2
  "3700 MVA 17KV :650KV Transformer "/LConn3 -- MPP1_3700MVA 17KV/RConn3 -- 185 MW/LConn3
  "500 MVA 17KV :650KV Transformer "/RConn3 -- 25 MW/LConn3 -- MPP2_500MVA 17KV/RConn3
  40 MW/LConn1 -- MPP3_800MVA 17KV/RConn1 -- 800 MVA 17KV :650KV Transformer/RConn1 -- Load Flow Bus4/LConn1
  MPP4_3800MVA 17KV/RConn1 -- 190 MW/LConn1 -- Load Flow Bus6/LConn1 -- 3800 MVA 17KV :650KV Transformer/RConn1
  "500 MVA 17KV :650KV Transformer "/LConn1 -- 1980 MVar/LConn1 -- TEST1-MPP2 187 km/LConn3
  CLP 1/RConn3 -- 990 MVar3/LConn3 -- CLP-CSG 103 km/RConn3
  Cs CSGN/LConn2 -- CLP-CSG 103 km/LConn2
  MPP4_3800MVA 17KV/RConn3 -- 190 MW/LConn3 -- 3800 MVA 17KV :650KV Transformer/RConn3
  "3700 MVA 17KV :650KV Transformer "/LConn1 -- Load Flow Bus/LConn1 -- 185 MW/LConn1 -- MPP1_3700MVA 17KV/RConn1
  CLP 1/LConn1 -- 4200 MVA 17KV :650KV Transformer/RConn1 -- Cs CLPN/RConn1 -- Cs CLPS/RConn1
  CLP 1/LConn2 -- 4200 MVA 17KV :650KV Transformer/RConn2 -- Cs CLPN/RConn2 -- Cs CLPS/RConn2
  3800 MVA 17KV :650KV Transformer/LConn2 -- MPP4-TEST2 96 km/LConn2
  "3700 MVA 17KV :650KV Transformer "/RConn1 -- MPP1-CLP 310 km/LConn1 -- Cs MPP1D/RConn1 -- 1320 MVar/LConn1 -- Load Flow Bus2/LConn1
  3800 MVA 17KV :650KV Transformer/LConn1 -- Load Flow Bus3/LConn1 -- MPP4-TEST2 96 km/LConn1
  "3700 MVA 17KV :650KV Transformer "/LConn2 -- 185 MW/LConn2 -- MPP1_3700MVA 17KV/RConn2
  MPP3-TEST2 111 km/RConn3 -- 660 MVar4/LConn1 -- MPP4-TEST2 96 km/RConn3 -- TEST2/LConn3
  TEST1-MPP2 187 km/RConn1 -- TEST 1/LConn3 -- TEST1-PNS 235 km/LConn3
  TEST2/RConn3 -- CLP-TEST2 288 km/LConn3
  MPP3-TEST2 111 km/RConn1 -- 660 MVar4/LConn3 -- MPP4-TEST2 96 km/RConn1 -- TEST2/LConn1
  Cs CLPS/LConn2 -- Cs AND/RConn2 -- CLP-TEST2 288 km/RConn2
  CLP-TEST2 288 km/RConn3 -- Cs CLPS/LConn3 -- Cs AND/RConn3
  800 MVA 17KV :650KV Transformer/LConn2 -- MPP3-TEST2 111 km/LConn2
  CSG 1/LConn3 -- Cs CSGN/RConn3
  MPP4_3800MVA 17KV/RConn2 -- 190 MW/LConn2 -- 3800 MVA 17KV :650KV Transformer/RConn2
  800 MVA 17KV :650KV Transformer/RConn2 -- 40 MW/LConn2 -- MPP3_800MVA 17KV/RConn2
  800 MVA 17KV :650KV Transformer/LConn1 -- MPP3-TEST2 111 km/LConn1
  MPP1-CLP 310 km/RConn1 -- Cs CLPN/LConn1
  MPP1-CLP 310 km/RConn3 -- Cs CLPN/LConn3
  TEST1-MPP2 187 km/LConn2 -- 1980 MVar/LConn2 -- "500 MVA 17KV :650KV Transformer "/LConn2
  TEST2/RConn1 -- Load Flow Bus5/LConn1 -- CLP-TEST2 288 km/LConn1
  MPP2_500MVA 17KV/RConn1 -- Load Flow Bus1/LConn1 -- 25 MW/LConn1 -- "500 MVA 17KV :650KV Transformer "/RConn1
  800 MVA 17KV :650KV Transformer/LConn3 -- MPP3-TEST2 111 km/LConn3
  MPP1-CLP 310 km/RConn2 -- Cs CLPN/LConn2
  CLP-CSG 103 km/RConn2 -- 990 MVar3/LConn2 -- CLP 1/RConn2
  CSG 1/LConn2 -- Cs CSGN/RConn2
  MPP3_800MVA 17KV/RConn3 -- 40 MW/LConn3 -- 800 MVA 17KV :650KV Transformer/RConn3
  CSG 1/LConn1 -- Cs CSGN/RConn1
  TEST2/RConn2 -- CLP-TEST2 288 km/LConn2
  3800 MVA 17KV :650KV Transformer/LConn3 -- MPP4-TEST2 96 km/LConn3
  Cs CSGN/LConn1 -- CLP-CSG 103 km/LConn1
  MPP5_4200MVA 17KV/RConn1 -- 210 MW/LConn1 -- 4200 MVA 17KV :650KV Transformer/LConn1 -- Load Flow Bus10/LConn1
  MPP5_4200MVA 17KV/RConn2 -- 210 MW/LConn2 -- 4200 MVA 17KV :650KV Transformer/LConn2
  MPP5_4200MVA 17KV/RConn3 -- 210 MW/LConn3 -- 4200 MVA 17KV :650KV Transformer/LConn3
  MPP6_490MVA 17KV/RConn1 -- 25 MW1/LConn1 -- 490 MVA 17KV :650KV Transformer/LConn1 -- Load Flow Bus12/LConn1
  MPP6_490MVA 17KV/RConn2 -- 25 MW1/LConn2 -- 490 MVA 17KV :650KV Transformer/LConn2
  MPP6_490MVA 17KV/RConn3 -- 25 MW1/LConn3 -- 490 MVA 17KV :650KV Transformer/LConn3
  Cs PNSM/LConn3 -- PNS3/RConn3
  Cs PNSM/LConn1 -- PNS3/RConn1
  Cs PNSM/LConn2 -- PNS3/RConn2
  Cs PNSN/RConn2 -- PNS3/LConn2
  PNS3/LConn3 -- Cs PNSN/RConn3
  Cs PNSN/RConn1 -- PNS3/LConn1 -- Load Flow Bus8/LConn1
  490 MVA 17KV :650KV Transformer/RConn1 -- 2310 MVar/LConn1 -- MPP6-CSG 186 km/LConn1
  490 MVA 17KV :650KV Transformer/RConn2 -- 2310 MVar/LConn2 -- MPP6-CSG 186 km/LConn2
  MPP6-CSG 186 km/RConn1 -- CSG 1/RConn1
  MPP6-CSG 186 km/RConn2 -- CSG 1/RConn2
  MPP6-CSG 186 km/RConn3 -- CSG 1/RConn3
  490 MVA 17KV :650KV Transformer/RConn3 -- 2310 MVar/LConn3 -- MPP6-CSG 186 km/LConn3
  SAT-a/RConn1 -- 660 MVar/LConn1 -- Cs SATS/RConn1
  SAT-b/RConn1 -- 660 MVar/LConn2 -- Cs SATS/RConn2
  SAT-c/RConn1 -- 660 MVar/LConn3 -- Cs SATS/RConn3
  Cs SATS/LConn3 -- " SAT-AND 129 km"/LConn3
  " SAT-AND 129 km"/LConn1 -- Cs SATS/LConn1
  Cs SATS/LConn2 -- " SAT-AND 129 km"/LConn2
  Cs PNSM/RConn1 -- TEST1-PNS 235 km/RConn1
  TEST1-PNS 235 km/RConn2 -- Cs PNSM/RConn2
  Cs PNSM/RConn3 -- TEST1-PNS 235 km/RConn3
  PNS-CON 260 km/LConn1 -- 990 MVar/LConn1 -- Cs PNSN/LConn1
  PNS-CON 260 km/LConn2 -- 990 MVar/LConn2 -- Cs PNSN/LConn2
  PNS-CON 260 km/LConn3 -- 990 MVar/LConn3 -- Cs PNSN/LConn3
  CON-a/RConn1 -- PNS-CON 260 km/RConn1
  CON-b/RConn1 -- PNS-CON 260 km/RConn2
  CON-c/RConn1 -- PNS-CON 260 km/RConn3
  AND1/RConn3 -- " SAT-AND 129 km"/RConn3
  AND1/RConn2 -- " SAT-AND 129 km"/RConn2
  AND1/RConn1 -- " SAT-AND 129 km"/RConn1
  Cs AND/LConn1 -- AND1/LConn1
  Cs AND/LConn3 -- Load Flow Bus11/LConn1 -- AND1/LConn3
  Cs AND/LConn2 -- AND1/LConn2
  TEST1-PNS 235 km/LConn1 -- TEST 1/LConn1 -- TEST1-MPP2 187 km/RConn3
  "3700 MVA 17KV :650KV Transformer "/RConn2 -- Cs MPP1D/RConn2 -- 1320 MVar/LConn2 -- MPP1-CLP 310 km/LConn2
  MPP1-CLP 310 km/LConn3 -- Cs MPP1D/RConn3 -- 1320 MVar/LConn3 -- "3700 MVA 17KV :650KV Transformer "/RConn3
  TEST 1/RConn1 -- Cs MPP1D/LConn1
  TEST 1/RConn2 -- Cs MPP1D/LConn2
  TEST 1/RConn3 -- Cs MPP1D/LConn3
